simulink model "SingleStreamSSR"  (R2025a)
settings: Solver=VariableStepAuto  StartTime=0.0  StopTime=4096  RelTol=1e-3
PreLoadFcn:
  | xmcCheckSlxPath(bdroot)
  | SSR4_init
InitFcn:
  | xmcCheckSlxPath(bdroot)
  | SSR4_init;
values from neighbouring files (symbols this model uses):
  N = 512    [SSR4_init.m]
  SHIFT_ACC = 15    [SSR4_init.m]
  Taps = NormalizeCoef(UTaps,32768)    [SSR4_init.m]
undefined symbols (not defined in the file or in its folder): FIR_MultiKernel_cin, FIR_MultiKernel_cincout, FIR_MultiKernel_cout, S, SingleStream, vsva2197, xcvc1902
libraries: aieBasic x40, aieUtilities x8, dspobslib x1, simulink x1, vmcUtilities x1
(part 2 of 3)

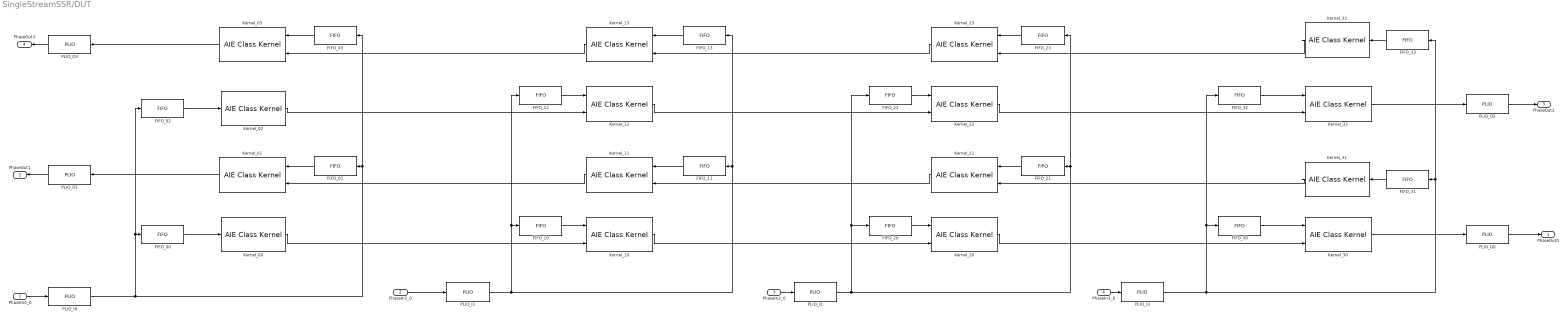
== system SingleStreamSSR/DUT ==
  PhaseIn0_0 : Inport
  PhaseIn1_0 : Inport  Port=2
  PhaseIn2_0 : Inport  Port=3
  PhaseIn3_0 : Inport  Port=4
  FIFO_00 : aieBasic/FIFO  FifoDepth=512  FIFOType=0  TileType=0  RowLocation=0  ColLocation=0  channel=0  blockJsonConstraints="[{\"type\":\"constraint\",\"constraintType\":\"location_fifo\",\"sid\":\"401\",\"lhs\":{\"type\":\"location\",\"templParam\":\"fifo\",\"args\":{\"type\":\"fifo\",\"name\":\"SingleStreamSSR/SSR4/FIFO_00\",\"sid\":\"401\"}},\"rhs\":{\"type\":\"fifogroup\",\"fifotype\":\"dma_fifo\",\"tiletype\":\"aie\",\"column\":{\"type\":\"evaluable\",\"expr\":\"25\",\"value\":25},\"row\":{\"type\":\"evaluable\",\"expr\":\"0\",\"value\":0},\"address\":{\"type\":\"evaluable\",\"expr\":\"0x0000\",\"value\":0},\"identifier\":\"0\",\"size\":{\"type\":\"evaluable\",\"expr\":\"512\",\"value\":512}},\"equality\":true}]"  deprecateConstraints=1
  FIFO_01 : aieBasic/FIFO  FifoDepth=512  FIFOType=0  TileType=0  RowLocation=0  ColLocation=0  channel=0  blockJsonConstraints="[{\"type\":\"constraint\",\"constraintType\":\"location_fifo\",\"sid\":\"404\",\"lhs\":{\"type\":\"location\",\"templParam\":\"fifo\",\"args\":{\"type\":\"fifo\",\"name\":\"SingleStreamSSR/SSR4/FIFO_01\",\"sid\":\"404\"}},\"rhs\":{\"type\":\"fifogroup\",\"fifotype\":\"dma_fifo\",\"tiletype\":\"aie\",\"column\":{\"type\":\"evaluable\",\"expr\":\"25\",\"value\":25},\"row\":{\"type\":\"evaluable\",\"expr\":\"1\",\"value\":1},\"address\":{\"type\":\"evaluable\",\"expr\":\"0x0000\",\"value\":0},\"identifier\":\"0\",\"size\":{\"type\":\"evaluable\",\"expr\":\"512\",\"value\":512}},\"equality\":true}]"  deprecateConstraints=1
  FIFO_02 : aieBasic/FIFO  FifoDepth=512  FIFOType=0  TileType=0  RowLocation=0  ColLocation=0  channel=0  blockJsonConstraints="[{\"type\":\"constraint\",\"constraintType\":\"location_fifo\",\"sid\":\"402\",\"lhs\":{\"type\":\"location\",\"templParam\":\"fifo\",\"args\":{\"type\":\"fifo\",\"name\":\"SingleStreamSSR/SSR4/FIFO_02\",\"sid\":\"402\"}},\"rhs\":{\"type\":\"fifogroup\",\"fifotype\":\"dma_fifo\",\"tiletype\":\"aie\",\"column\":{\"type\":\"evaluable\",\"expr\":\"25\",\"value\":25},\"row\":{\"type\":\"evaluable\",\"expr\":\"2\",\"value\":2},\"address\":{\"type\":\"evaluable\",\"expr\":\"0x0000\",\"value\":0},\"identifier\":\"0\",\"size\":{\"type\":\"evaluable\",\"expr\":\"512\",\"value\":512}},\"equality\":true}]"  deprecateConstraints=1
  FIFO_03 : aieBasic/FIFO  FifoDepth=512  FIFOType=0  TileType=0  RowLocation=0  ColLocation=0  channel=0  blockJsonConstraints="[{\"type\":\"constraint\",\"constraintType\":\"location_fifo\",\"sid\":\"403\",\"lhs\":{\"type\":\"location\",\"templParam\":\"fifo\",\"args\":{\"type\":\"fifo\",\"name\":\"SingleStreamSSR/SSR4/FIFO_03\",\"sid\":\"403\"}},\"rhs\":{\"type\":\"fifogroup\",\"fifotype\":\"dma_fifo\",\"tiletype\":\"aie\",\"column\":{\"type\":\"evaluable\",\"expr\":\"25\",\"value\":25},\"row\":{\"type\":\"evaluable\",\"expr\":\"3\",\"value\":3},\"address\":{\"type\":\"evaluable\",\"expr\":\"0x0000\",\"value\":0},\"identifier\":\"0\",\"size\":{\"type\":\"evaluable\",\"expr\":\"512\",\"value\":512}},\"equality\":true}]"  deprecateConstraints=1
  FIFO_10 : aieBasic/FIFO  FifoDepth=512  FIFOType=0  TileType=0  RowLocation=0  ColLocation=0  channel=0  blockJsonConstraints="[{\"type\":\"constraint\",\"constraintType\":\"location_fifo\",\"sid\":\"405\",\"lhs\":{\"type\":\"location\",\"templParam\":\"fifo\",\"args\":{\"type\":\"fifo\",\"name\":\"SingleStreamSSR/SSR4/FIFO_10\",\"sid\":\"405\"}},\"rhs\":{\"type\":\"fifogroup\",\"fifotype\":\"dma_fifo\",\"tiletype\":\"aie\",\"column\":{\"type\":\"evaluable\",\"expr\":\"26\",\"value\":26},\"row\":{\"type\":\"evaluable\",\"expr\":\"0\",\"value\":0},\"address\":{\"type\":\"evaluable\",\"expr\":\"0x0000\",\"value\":0},\"identifier\":\"0\",\"size\":{\"type\":\"evaluable\",\"expr\":\"512\",\"value\":512}},\"equality\":true}]"  deprecateConstraints=1
  FIFO_11 : aieBasic/FIFO  FifoDepth=512  FIFOType=0  TileType=0  RowLocation=0  ColLocation=0  channel=0  blockJsonConstraints="[{\"type\":\"constraint\",\"constraintType\":\"location_fifo\",\"sid\":\"407\",\"lhs\":{\"type\":\"location\",\"templParam\":\"fifo\",\"args\":{\"type\":\"fifo\",\"name\":\"SingleStreamSSR/SSR4/FIFO_11\",\"sid\":\"407\"}},\"rhs\":{\"type\":\"fifogroup\",\"fifotype\":\"dma_fifo\",\"tiletype\":\"aie\",\"column\":{\"type\":\"evaluable\",\"expr\":\"26\",\"value\":26},\"row\":{\"type\":\"evaluable\",\"expr\":\"1\",\"value\":1},\"address\":{\"type\":\"evaluable\",\"expr\":\"0x0000\",\"value\":0},\"identifier\":\"0\",\"size\":{\"type\":\"evaluable\",\"expr\":\"512\",\"value\":512}},\"equality\":true}]"  deprecateConstraints=1
  FIFO_12 : aieBasic/FIFO  FifoDepth=512  FIFOType=0  TileType=0  RowLocation=0  ColLocation=0  channel=0  blockJsonConstraints="[{\"type\":\"constraint\",\"constraintType\":\"location_fifo\",\"sid\":\"406\",\"lhs\":{\"type\":\"location\",\"templParam\":\"fifo\",\"args\":{\"type\":\"fifo\",\"name\":\"SingleStreamSSR/SSR4/FIFO_12\",\"sid\":\"406\"}},\"rhs\":{\"type\":\"fifogroup\",\"fifotype\":\"dma_fifo\",\"tiletype\":\"aie\",\"column\":{\"type\":\"evaluable\",\"expr\":\"26\",\"value\":26},\"row\":{\"type\":\"evaluable\",\"expr\":\"2\",\"value\":2},\"address\":{\"type\":\"evaluable\",\"expr\":\"0x0000\",\"value\":0},\"identifier\":\"0\",\"size\":{\"type\":\"evaluable\",\"expr\":\"512\",\"value\":512}},\"equality\":true}]"  deprecateConstraints=1
  FIFO_13 : aieBasic/FIFO  FifoDepth=512  FIFOType=0  TileType=0  RowLocation=0  ColLocation=0  channel=0  blockJsonConstraints="[{\"type\":\"constraint\",\"constraintType\":\"location_fifo\",\"sid\":\"408\",\"lhs\":{\"type\":\"location\",\"templParam\":\"fifo\",\"args\":{\"type\":\"fifo\",\"name\":\"SingleStreamSSR/SSR4/FIFO_13\",\"sid\":\"408\"}},\"rhs\":{\"type\":\"fifogroup\",\"fifotype\":\"dma_fifo\",\"tiletype\":\"aie\",\"column\":{\"type\":\"evaluable\",\"expr\":\"26\",\"value\":26},\"row\":{\"type\":\"evaluable\",\"expr\":\"3\",\"value\":3},\"address\":{\"type\":\"evaluable\",\"expr\":\"0x0000\",\"value\":0},\"identifier\":\"0\",\"size\":{\"type\":\"evaluable\",\"expr\":\"512\",\"value\":512}},\"equality\":true}]"  deprecateConstraints=1
  FIFO_20 : aieBasic/FIFO  FifoDepth=512  FIFOType=0  TileType=0  RowLocation=0  ColLocation=0  channel=0  blockJsonConstraints="[{\"type\":\"constraint\",\"constraintType\":\"location_fifo\",\"sid\":\"409\",\"lhs\":{\"type\":\"location\",\"templParam\":\"fifo\",\"args\":{\"type\":\"fifo\",\"name\":\"SingleStreamSSR/SSR4/FIFO_20\",\"sid\":\"409\"}},\"rhs\":{\"type\":\"fifogroup\",\"fifotype\":\"dma_fifo\",\"tiletype\":\"aie\",\"column\":{\"type\":\"evaluable\",\"expr\":\"27\",\"value\":27},\"row\":{\"type\":\"evaluable\",\"expr\":\"0\",\"value\":0},\"address\":{\"type\":\"evaluable\",\"expr\":\"0x0000\",\"value\":0},\"identifier\":\"0\",\"size\":{\"type\":\"evaluable\",\"expr\":\"512\",\"value\":512}},\"equality\":true}]"  deprecateConstraints=1
  FIFO_21 : aieBasic/FIFO  FifoDepth=512  FIFOType=0  TileType=0  RowLocation=0  ColLocation=0  channel=0  blockJsonConstraints="[{\"type\":\"constraint\",\"constraintType\":\"location_fifo\",\"sid\":\"412\",\"lhs\":{\"type\":\"location\",\"templParam\":\"fifo\",\"args\":{\"type\":\"fifo\",\"name\":\"SingleStreamSSR/SSR4/FIFO_21\",\"sid\":\"412\"}},\"rhs\":{\"type\":\"fifogroup\",\"fifotype\":\"dma_fifo\",\"tiletype\":\"aie\",\"column\":{\"type\":\"evaluable\",\"expr\":\"27\",\"value\":27},\"row\":{\"type\":\"evaluable\",\"expr\":\"1\",\"value\":1},\"address\":{\"type\":\"evaluable\",\"expr\":\"0x0000\",\"value\":0},\"identifier\":\"0\",\"size\":{\"type\":\"evaluable\",\"expr\":\"512\",\"value\":512}},\"equality\":true}]"  deprecateConstraints=1
  FIFO_22 : aieBasic/FIFO  FifoDepth=512  FIFOType=0  TileType=0  RowLocation=0  ColLocation=0  channel=0  blockJsonConstraints="[{\"type\":\"constraint\",\"constraintType\":\"location_fifo\",\"sid\":\"410\",\"lhs\":{\"type\":\"location\",\"templParam\":\"fifo\",\"args\":{\"type\":\"fifo\",\"name\":\"SingleStreamSSR/SSR4/FIFO_22\",\"sid\":\"410\"}},\"rhs\":{\"type\":\"fifogroup\",\"fifotype\":\"dma_fifo\",\"tiletype\":\"aie\",\"column\":{\"type\":\"evaluable\",\"expr\":\"27\",\"value\":27},\"row\":{\"type\":\"evaluable\",\"expr\":\"2\",\"value\":2},\"address\":{\"type\":\"evaluable\",\"expr\":\"0x0000\",\"value\":0},\"identifier\":\"0\",\"size\":{\"type\":\"evaluable\",\"expr\":\"512\",\"value\":512}},\"equality\":true}]"  deprecateConstraints=1
  FIFO_23 : aieBasic/FIFO  FifoDepth=512  FIFOType=0  TileType=0  RowLocation=0  ColLocation=0  channel=0  blockJsonConstraints="[{\"type\":\"constraint\",\"constraintType\":\"location_fifo\",\"sid\":\"411\",\"lhs\":{\"type\":\"location\",\"templParam\":\"fifo\",\"args\":{\"type\":\"fifo\",\"name\":\"SingleStreamSSR/SSR4/FIFO_23\",\"sid\":\"411\"}},\"rhs\":{\"type\":\"fifogroup\",\"fifotype\":\"dma_fifo\",\"tiletype\":\"aie\",\"column\":{\"type\":\"evaluable\",\"expr\":\"27\",\"value\":27},\"row\":{\"type\":\"evaluable\",\"expr\":\"3\",\"value\":3},\"address\":{\"type\":\"evaluable\",\"expr\":\"0x0000\",\"value\":0},\"identifier\":\"0\",\"size\":{\"type\":\"evaluable\",\"expr\":\"512\",\"value\":512}},\"equality\":true}]"  deprecateConstraints=1
  FIFO_30 : aieBasic/FIFO  FifoDepth=512  FIFOType=0  TileType=0  RowLocation=0  ColLocation=0  channel=0  blockJsonConstraints="[{\"type\":\"constraint\",\"constraintType\":\"location_fifo\",\"sid\":\"413\",\"lhs\":{\"type\":\"location\",\"templParam\":\"fifo\",\"args\":{\"type\":\"fifo\",\"name\":\"SingleStreamSSR/SSR4/FIFO_30\",\"sid\":\"413\"}},\"rhs\":{\"type\":\"fifogroup\",\"fifotype\":\"dma_fifo\",\"tiletype\":\"aie\",\"column\":{\"type\":\"evaluable\",\"expr\":\"28\",\"value\":28},\"row\":{\"type\":\"evaluable\",\"expr\":\"0\",\"value\":0},\"address\":{\"type\":\"evaluable\",\"expr\":\"0x0000\",\"value\":0},\"identifier\":\"0\",\"size\":{\"type\":\"evaluable\",\"expr\":\"512\",\"value\":512}},\"equality\":true}]"  deprecateConstraints=1
  FIFO_31 : aieBasic/FIFO  FifoDepth=512  FIFOType=0  TileType=0  RowLocation=0  ColLocation=0  channel=0  blockJsonConstraints="[{\"type\":\"constraint\",\"constraintType\":\"location_fifo\",\"sid\":\"416\",\"lhs\":{\"type\":\"location\",\"templParam\":\"fifo\",\"args\":{\"type\":\"fifo\",\"name\":\"SingleStreamSSR/SSR4/FIFO_31\",\"sid\":\"416\"}},\"rhs\":{\"type\":\"fifogroup\",\"fifotype\":\"dma_fifo\",\"tiletype\":\"aie\",\"column\":{\"type\":\"evaluable\",\"expr\":\"28\",\"value\":28},\"row\":{\"type\":\"evaluable\",\"expr\":\"1\",\"value\":1},\"address\":{\"type\":\"evaluable\",\"expr\":\"0x0000\",\"value\":0},\"identifier\":\"0\",\"size\":{\"type\":\"evaluable\",\"expr\":\"512\",\"value\":512}},\"equality\":true}]"  deprecateConstraints=1
  FIFO_32 : aieBasic/FIFO  FifoDepth=512  FIFOType=0  TileType=0  RowLocation=0  ColLocation=0  channel=0  blockJsonConstraints="[{\"type\":\"constraint\",\"constraintType\":\"location_fifo\",\"sid\":\"414\",\"lhs\":{\"type\":\"location\",\"templParam\":\"fifo\",\"args\":{\"type\":\"fifo\",\"name\":\"SingleStreamSSR/SSR4/FIFO_32\",\"sid\":\"414\"}},\"rhs\":{\"type\":\"fifogroup\",\"fifotype\":\"dma_fifo\",\"tiletype\":\"aie\",\"column\":{\"type\":\"evaluable\",\"expr\":\"28\",\"value\":28},\"row\":{\"type\":\"evaluable\",\"expr\":\"2\",\"value\":2},\"address\":{\"type\":\"evaluable\",\"expr\":\"0x0000\",\"value\":0},\"identifier\":\"0\",\"size\":{\"type\":\"evaluable\",\"expr\":\"512\",\"value\":512}},\"equality\":true}]"  deprecateConstraints=1
  FIFO_33 : aieBasic/FIFO  FifoDepth=512  FIFOType=0  TileType=0  RowLocation=0  ColLocation=0  channel=0  blockJsonConstraints="[{\"type\":\"constraint\",\"constraintType\":\"location_fifo\",\"sid\":\"415\",\"lhs\":{\"type\":\"location\",\"templParam\":\"fifo\",\"args\":{\"type\":\"fifo\",\"name\":\"SingleStreamSSR/SSR4/FIFO_33\",\"sid\":\"415\"}},\"rhs\":{\"type\":\"fifogroup\",\"fifotype\":\"dma_fifo\",\"tiletype\":\"aie\",\"column\":{\"type\":\"evaluable\",\"expr\":\"28\",\"value\":28},\"row\":{\"type\":\"evaluable\",\"expr\":\"3\",\"value\":3},\"address\":{\"type\":\"evaluable\",\"expr\":\"0x0000\",\"value\":0},\"identifier\":\"0\",\"size\":{\"type\":\"evaluable\",\"expr\":\"512\",\"value\":512}},\"equality\":true}]"  deprecateConstraints=1
  Kernel_00 : aieBasic/AIE Class Kernel  KernelAllAttrs=|  PortNames={'sin'; 'cout'}  PortSerializedTypes={'{P{Tinput_stream{1{t{Scint16}}}}}'; '{P{Toutput_cascade{2{t{Scacc48}}{t{Bv}}}}}'}  PortWindowSizes={0.000000000000000000e+00; 0.000000000000000000e+00}  PortWindowMargins={0.000000000000000000e+00; 0.000000000000000000e+00}  PortSynchronicities={'auto', 'auto'}  PortSignalSizes={0.000000000000000000e+00; 5.120000000000000000e+02}  ClassTemplateSpecKind=implicit  ClassTemplateParamNames={'NSamples'; 'ShiftAcc'}  ClassTemplateParamKinds={'nontype'; 'nontype'}  ClassTemplateParamTypes={'int'; 'int'}  ClassTemplateParamValues={'512', '15'}  ClassCtorParamNames={'taps'; 'Delay'}  ClassCtorParamSerializedTypes={'{R{Q1{C{Scint16}8}}}'; '{Q1{Bi32}}'}  ClassCtorParamValues={'[-54-21i -121-233i 102-525i 237-96i 8773-2748i 1454+497i 342+439i 14+121i]', '0'}  ClassIndex=1  ClassCtorIndex=1  ClassTabVisible=on  ClassTemplateParamsVisible=on  ClassCtorDeclVisible=on  ClassCtorParamsVisible=on  FunctionTabVisible=on  FunctionDecl=|  PortAttrs={ 'input', 'sin', 'input_stream_cint16 *', '', '0', '', ''; 'output', 'cout', 'output_cascade< cacc48, void > *', '', '', '', 'N' }  PortAttrsEnables={'off', 'off', 'off', 'off', 'off', 'off', 'off';'off', 'off', 'off', 'off', 'off', 'off', 'on'}  SampleTime=-1  ClassDeclTypeOptions=|  ClassDecl=|  ClassTemplateParams={ 'NSamples', 'int', 'BURST_LENGTH'; 'ShiftAcc', 'int', 'SHIFT_ACC' }  ClassTemplateParamsEnables={'off', 'off', 'on';'off', 'off', 'on'}  ClassCtorDeclTypeOptions=C[1 1]@t70@FIR_MultiKernel_cout(cint16 const ( & taps ) [ 8 ], int32 const Delay)  ClassCtorDecl=FIR_MultiKernel_cout(cint16 const ( & taps ) [ 8 ], int32 const Delay)  ClassCtorParams={ 'taps', 'cint16 const ( &) [ 8 ]', 'phi_0'; 'Delay', 'int32 const', '0' }  KernelHeaderFile=FirSingleStream.h  KernelClassName=SingleStream::FIR_MultiKernel_cout  KernelFunction=filter  KernelSourceFile=FirSingleStream.cpp  KernelSearchPaths={'$SRC', '$SRC/aie_kernels'}  PreProcOptions={}  blockJsonConstraints="{\"type\":\"constraint\",\"constraintType\":\"location_kernel\",\"sid\":\"386\",\"lhs\":{\"type\":\"location\",\"templParam\":\"kernel\",\"args\":{\"type\":\"kernel\",\"name\":\"SingleStreamSSR/SSR4/Kernel_00\",\"sid\":\"386\"}},\"rhs\":{\"type\":\"tile\",\"args\":[{\"type\":\"evaluable\",\"expr\":\"25\",\"value\":25},{\"type\":\"evaluable\",\"expr\":\"0\",\"value\":0}]},\"equality\":true}"
      KernelAllAttrs=|
      | s[12;12;9;9;19;14;21;23;21;23;24;21;15;17;12;24;26;26;26;27;28;9;21;23;23;23;24;25;14;19;19;29]@FunctionNameDeclFileNamePortNamesPortTypesPortSerializedTypesPortDirectionsPortWindowSizeEnablesPortWindowMarginEnablesPortBufferSizeEnablesPortBufferMarginEnablesPortSynchronicityEnablesPortSignalSizeEnablesPortBufferSizesPortBufferMarginsFunctionDeclFunctionTemplateSpecKindFunctionTemplateParamNamesFunctionTemplateParamKindsFunctionTemplateParamTypesFunctionTemplateParamValuesFunctionTemplateParamEnablesClassDeclClassTemplateSpecKindClassTemplateParamNamesClassTemplateParamKindsClassTemplateParamTypesClassTemplateParamValuesClassTemplateParamEnablesClassCtorDeclsClassCtorParamNamesClassCtorParamTypesClassCtorParamSerializedTypes[1 1]@C[32 1]@t6@filtert39@../../src/aie_kernels/FirSingleStream.hC[2 1]@t3@sint4@coutC[2 1]@t21@input_stream_cint16 *t32@output_cascade< cacc48, void > *C[2 1]@t33@{P{Tinput_stream{1{t{Scint16}}}}}t42@{P{Toutput_cascade{2{t{Scacc48}}{t{Bv}}}}}C[2 1]@t5@inputt6@outputC[2 1]@l0@l0@C[2 1]@l0@l0@C[2 1]@l0@l0@C[2 1]@l0@l0@C[2 1]@l0@l0@C[2 1]@l0@l1@C[2 1]@nnC[2 1]@nnt169@namespace SingleStream {
      | template < int NSamples, int ShiftAcc > 
      | void FIR_MultiKernel_cout::
      | filter(input_stream_cint16 * sin, output_cascade< cacc48, void > * cout);
      | }t4@nonee[0 1]@e[0 1]@e[0 1]@e[0 1]@e[0 1]@t94@namespace SingleStream {
      | template < int NSamples, int ShiftAcc > class FIR_MultiKernel_cout;
      | }t8@implicitC[2 1]@t8@NSamplest8@ShiftAccC[2 1]@t7@nontypet7@nontypeC[2 1]@t3@intt3@intC[2 1]@nnC[2 1]@l1@l1@C[1 1]@t70@FIR_MultiKernel_cout(cint16 const ( & taps ) [ 8 ], int32 const Delay)C[1 1]@C[2 1]@t4@tapst5@DelayC[1 1]@C[2 1]@t23@cint16 const ( &) [ 8 ]t11@int32 constC[1 1]@C[2 1]@t20@{R{Q1{C{Scint16}8}}}t10@{Q1{Bi32}}
      FunctionDecl=|
      | namespace SingleStream {
      | template < int NSamples, int ShiftAcc > 
      | void FIR_MultiKernel_cout::
      | filter(input_stream_cint16 * sin, output_cascade< cacc48, void > * cout);
      | }
      ClassDeclTypeOptions=|
      | C[1 1]@t94@namespace SingleStream {
      | template < int NSamples, int ShiftAcc > class FIR_MultiKernel_cout;
      | }
      ClassDecl=|
      | namespace SingleStream {
      | template < int NSamples, int ShiftAcc > class FIR_MultiKernel_cout;
      | }
  Kernel_01 : aieBasic/AIE Class Kernel  KernelAllAttrs=|  PortNames={'sin'; 'cin'; 'sout'}  PortSerializedTypes={'{P{Tinput_stream{1{t{Scint16}}}}}'; '{P{Tinput_cascade{2{t{Scacc48}}{t{Bv}}}}}'; '{P{Toutput_stream{1{t{Scint16}}}}}'}  PortWindowSizes={0.000000000000000000e+00; 0.000000000000000000e+00; 0.000000000000000000e+00}  PortWindowMargins={0.000000000000000000e+00; 0.000000000000000000e+00; 0.000000000000000000e+00}  PortSynchronicities={'auto', 'auto', 'auto'}  PortSignalSizes={0.000000000000000000e+00; 0.000000000000000000e+00; 5.120000000000000000e+02}  ClassTemplateSpecKind=implicit  ClassTemplateParamNames={'NSamples'; 'ShiftAcc'}  ClassTemplateParamKinds={'nontype'; 'nontype'}  ClassTemplateParamTypes={'int'; 'int'}  ClassTemplateParamValues={'512', '15'}  ClassCtorParamNames={'taps'; 'Delay'}  ClassCtorParamSerializedTypes={'{R{Q1{C{Scint16}8}}}'; '{Q1{Bi32}}'}  ClassCtorParamValues={'[14-121i 342-439i 1454-497i 8773+2748i 237+96i 102+525i -121+233i -54+21i]', '1'}  ClassIndex=1  ClassCtorIndex=1  ClassTabVisible=on  ClassTemplateParamsVisible=on  ClassCtorDeclVisible=on  ClassCtorParamsVisible=on  FunctionTabVisible=on  FunctionDecl=|  PortAttrs={ 'input', 'sin', 'input_stream_cint16 *', '', '0', '', ''; 'input', 'cin', 'input_cascade< cacc48, void > *', '', '0', '', ''; 'output', 'sout', 'output_stream_cint16 *', '', '', '', 'N' }  PortAttrsEnables={'off', 'off', 'off', 'off', 'off', 'off', 'off';'off', 'off', 'off', 'off', 'off', 'off', 'off';'off', 'off', 'off', 'off', 'off', 'off', 'on'}  SampleTime=-1  ClassDeclTypeOptions=|  ClassDecl=|  ClassTemplateParams={ 'NSamples', 'int', 'BURST_LENGTH'; 'ShiftAcc', 'int', 'SHIFT_ACC' }  ClassTemplateParamsEnables={'off', 'off', 'on';'off', 'off', 'on'}  ClassCtorDeclTypeOptions=C[1 1]@t69@FIR_MultiKernel_cin(cint16 const ( & taps ) [ 8 ], int32 const Delay)  ClassCtorDecl=FIR_MultiKernel_cin(cint16 const ( & taps ) [ 8 ], int32 const Delay)  ClassCtorParams={ 'taps', 'cint16 const ( &) [ 8 ]', 'phi_3'; 'Delay', 'int32 const', '1' }  KernelHeaderFile=FirSingleStream.h  KernelClassName=SingleStream::FIR_MultiKernel_cin  KernelFunction=filter  KernelSourceFile=FirSingleStream.cpp  KernelSearchPaths={'$SRC', '$SRC/aie_kernels'}  PreProcOptions={}  blockJsonConstraints=[]
      KernelAllAttrs=|
      | s[12;12;9;9;19;14;21;23;21;23;24;21;15;17;12;24;26;26;26;27;28;9;21;23;23;23;24;25;14;19;19;29]@FunctionNameDeclFileNamePortNamesPortTypesPortSerializedTypesPortDirectionsPortWindowSizeEnablesPortWindowMarginEnablesPortBufferSizeEnablesPortBufferMarginEnablesPortSynchronicityEnablesPortSignalSizeEnablesPortBufferSizesPortBufferMarginsFunctionDeclFunctionTemplateSpecKindFunctionTemplateParamNamesFunctionTemplateParamKindsFunctionTemplateParamTypesFunctionTemplateParamValuesFunctionTemplateParamEnablesClassDeclClassTemplateSpecKindClassTemplateParamNamesClassTemplateParamKindsClassTemplateParamTypesClassTemplateParamValuesClassTemplateParamEnablesClassCtorDeclsClassCtorParamNamesClassCtorParamTypesClassCtorParamSerializedTypes[1 1]@C[32 1]@t6@filtert39@../../src/aie_kernels/FirSingleStream.hC[3 1]@t3@sint3@cint4@soutC[3 1]@t21@input_stream_cint16 *t31@input_cascade< cacc48, void > *t22@output_stream_cint16 *C[3 1]@t33@{P{Tinput_stream{1{t{Scint16}}}}}t41@{P{Tinput_cascade{2{t{Scacc48}}{t{Bv}}}}}t34@{P{Toutput_stream{1{t{Scint16}}}}}C[3 1]@t5@inputt5@inputt6@outputC[3 1]@l0@l0@l0@C[3 1]@l0@l0@l0@C[3 1]@l0@l0@l0@C[3 1]@l0@l0@l0@C[3 1]@l0@l0@l0@C[3 1]@l0@l0@l1@C[3 1]@nnnC[3 1]@nnnt195@namespace SingleStream {
      | template < int NSamples, int ShiftAcc > 
      | void FIR_MultiKernel_cin::
      | filter(input_stream_cint16 * sin, input_cascade< cacc48, void > * cin, output_stream_cint16 * sout);
      | }t4@nonee[0 1]@e[0 1]@e[0 1]@e[0 1]@e[0 1]@t93@namespace SingleStream {
      | template < int NSamples, int ShiftAcc > class FIR_MultiKernel_cin;
      | }t8@implicitC[2 1]@t8@NSamplest8@ShiftAccC[2 1]@t7@nontypet7@nontypeC[2 1]@t3@intt3@intC[2 1]@nnC[2 1]@l1@l1@C[1 1]@t69@FIR_MultiKernel_cin(cint16 const ( & taps ) [ 8 ], int32 const Delay)C[1 1]@C[2 1]@t4@tapst5@DelayC[1 1]@C[2 1]@t23@cint16 const ( &) [ 8 ]t11@int32 constC[1 1]@C[2 1]@t20@{R{Q1{C{Scint16}8}}}t10@{Q1{Bi32}}
      FunctionDecl=|
      | namespace SingleStream {
      | template < int NSamples, int ShiftAcc > 
      | void FIR_MultiKernel_cin::
      | filter(input_stream_cint16 * sin, input_cascade< cacc48, void > * cin, output_stream_cint16 * sout);
      | }
      ClassDeclTypeOptions=|
      | C[1 1]@t93@namespace SingleStream {
      | template < int NSamples, int ShiftAcc > class FIR_MultiKernel_cin;
      | }
      ClassDecl=|
      | namespace SingleStream {
      | template < int NSamples, int ShiftAcc > class FIR_MultiKernel_cin;
      | }
  Kernel_02 : aieBasic/AIE Class Kernel  KernelAllAttrs=|  PortNames={'sin'; 'cout'}  PortSerializedTypes={'{P{Tinput_stream{1{t{Scint16}}}}}'; '{P{Toutput_cascade{2{t{Scacc48}}{t{Bv}}}}}'}  PortWindowSizes={0.000000000000000000e+00; 0.000000000000000000e+00}  PortWindowMargins={0.000000000000000000e+00; 0.000000000000000000e+00}  PortSynchronicities={'auto', 'auto'}  PortSignalSizes={0.000000000000000000e+00; 5.120000000000000000e+02}  ClassTemplateSpecKind=implicit  ClassTemplateParamNames={'NSamples'; 'ShiftAcc'}  ClassTemplateParamKinds={'nontype'; 'nontype'}  ClassTemplateParamTypes={'int'; 'int'}  ClassTemplateParamValues={'512', '15'}  ClassCtorParamNames={'taps'; 'Delay'}  ClassCtorParamSerializedTypes={'{R{Q1{C{Scint16}8}}}'; '{Q1{Bi32}}'}  ClassCtorParamValues={'[-21+26i 146-91i 1183+239i 4086+5221i 248-2878i 237-54i -160+111i -83-21i]', '1'}  ClassIndex=1  ClassCtorIndex=1  ClassTabVisible=on  ClassTemplateParamsVisible=on  ClassCtorDeclVisible=on  ClassCtorParamsVisible=on  FunctionTabVisible=on  FunctionDecl=|  PortAttrs={ 'input', 'sin', 'input_stream_cint16 *', '', '0', '', ''; 'output', 'cout', 'output_cascade< cacc48, void > *', '', '', '', 'N' }  PortAttrsEnables={'off', 'off', 'off', 'off', 'off', 'off', 'off';'off', 'off', 'off', 'off', 'off', 'off', 'on'}  SampleTime=-1  ClassDeclTypeOptions=|  ClassDecl=|  ClassTemplateParams={ 'NSamples', 'int', 'BURST_LENGTH'; 'ShiftAcc', 'int', 'SHIFT_ACC' }  ClassTemplateParamsEnables={'off', 'off', 'on';'off', 'off', 'on'}  ClassCtorDeclTypeOptions=C[1 1]@t70@FIR_MultiKernel_cout(cint16 const ( & taps ) [ 8 ], int32 const Delay)  ClassCtorDecl=FIR_MultiKernel_cout(cint16 const ( & taps ) [ 8 ], int32 const Delay)  ClassCtorParams={ 'taps', 'cint16 const ( &) [ 8 ]', 'phi_2'; 'Delay', 'int32 const', '1' }  KernelHeaderFile=FirSingleStream.h  KernelClassName=SingleStream::FIR_MultiKernel_cout  KernelFunction=filter  KernelSourceFile=FirSingleStream.cpp  KernelSearchPaths={'$SRC', '$SRC/aie_kernels'}  PreProcOptions={}  blockJsonConstraints="{\"type\":\"constraint\",\"constraintType\":\"location_kernel\",\"sid\":\"341\",\"lhs\":{\"type\":\"location\",\"templParam\":\"kernel\",\"args\":{\"type\":\"kernel\",\"name\":\"SingleStreamSSR/SSR4/Kernel_02\",\"sid\":\"341\"}},\"rhs\":{\"type\":\"tile\",\"args\":[{\"type\":\"evaluable\",\"expr\":\"25\",\"value\":25},{\"type\":\"evaluable\",\"expr\":\"2\",\"value\":2}]},\"equality\":true}"
      KernelAllAttrs=|
      | s[12;12;9;9;19;14;21;23;21;23;24;21;15;17;12;24;26;26;26;27;28;9;21;23;23;23;24;25;14;19;19;29]@FunctionNameDeclFileNamePortNamesPortTypesPortSerializedTypesPortDirectionsPortWindowSizeEnablesPortWindowMarginEnablesPortBufferSizeEnablesPortBufferMarginEnablesPortSynchronicityEnablesPortSignalSizeEnablesPortBufferSizesPortBufferMarginsFunctionDeclFunctionTemplateSpecKindFunctionTemplateParamNamesFunctionTemplateParamKindsFunctionTemplateParamTypesFunctionTemplateParamValuesFunctionTemplateParamEnablesClassDeclClassTemplateSpecKindClassTemplateParamNamesClassTemplateParamKindsClassTemplateParamTypesClassTemplateParamValuesClassTemplateParamEnablesClassCtorDeclsClassCtorParamNamesClassCtorParamTypesClassCtorParamSerializedTypes[1 1]@C[32 1]@t6@filtert39@../../src/aie_kernels/FirSingleStream.hC[2 1]@t3@sint4@coutC[2 1]@t21@input_stream_cint16 *t32@output_cascade< cacc48, void > *C[2 1]@t33@{P{Tinput_stream{1{t{Scint16}}}}}t42@{P{Toutput_cascade{2{t{Scacc48}}{t{Bv}}}}}C[2 1]@t5@inputt6@outputC[2 1]@l0@l0@C[2 1]@l0@l0@C[2 1]@l0@l0@C[2 1]@l0@l0@C[2 1]@l0@l0@C[2 1]@l0@l1@C[2 1]@nnC[2 1]@nnt169@namespace SingleStream {
      | template < int NSamples, int ShiftAcc > 
      | void FIR_MultiKernel_cout::
      | filter(input_stream_cint16 * sin, output_cascade< cacc48, void > * cout);
      | }t4@nonee[0 1]@e[0 1]@e[0 1]@e[0 1]@e[0 1]@t94@namespace SingleStream {
      | template < int NSamples, int ShiftAcc > class FIR_MultiKernel_cout;
      | }t8@implicitC[2 1]@t8@NSamplest8@ShiftAccC[2 1]@t7@nontypet7@nontypeC[2 1]@t3@intt3@intC[2 1]@nnC[2 1]@l1@l1@C[1 1]@t70@FIR_MultiKernel_cout(cint16 const ( & taps ) [ 8 ], int32 const Delay)C[1 1]@C[2 1]@t4@tapst5@DelayC[1 1]@C[2 1]@t23@cint16 const ( &) [ 8 ]t11@int32 constC[1 1]@C[2 1]@t20@{R{Q1{C{Scint16}8}}}t10@{Q1{Bi32}}
      FunctionDecl=|
      | namespace SingleStream {
      | template < int NSamples, int ShiftAcc > 
      | void FIR_MultiKernel_cout::
      | filter(input_stream_cint16 * sin, output_cascade< cacc48, void > * cout);
      | }
      ClassDeclTypeOptions=|
      | C[1 1]@t94@namespace SingleStream {
      | template < int NSamples, int ShiftAcc > class FIR_MultiKernel_cout;
      | }
      ClassDecl=|
      | namespace SingleStream {
      | template < int NSamples, int ShiftAcc > class FIR_MultiKernel_cout;
      | }
  Kernel_03 : aieBasic/AIE Class Kernel  KernelAllAttrs=|  PortNames={'sin'; 'cin'; 'sout'}  PortSerializedTypes={'{P{Tinput_stream{1{t{Scint16}}}}}'; '{P{Tinput_cascade{2{t{Scacc48}}{t{Bv}}}}}'; '{P{Toutput_stream{1{t{Scint16}}}}}'}  PortWindowSizes={0.000000000000000000e+00; 0.000000000000000000e+00; 0.000000000000000000e+00}  PortWindowMargins={0.000000000000000000e+00; 0.000000000000000000e+00; 0.000000000000000000e+00}  PortSynchronicities={'auto', 'auto', 'auto'}  PortSignalSizes={0.000000000000000000e+00; 0.000000000000000000e+00; 5.120000000000000000e+02}  ClassTemplateSpecKind=implicit  ClassTemplateParamNames={'NSamples'; 'ShiftAcc'}  ClassTemplateParamKinds={'nontype'; 'nontype'}  ClassTemplateParamTypes={'int'; 'int'}  ClassTemplateParamValues={'512', '15'}  ClassCtorParamNames={'taps'; 'Delay'}  ClassCtorParamSerializedTypes={'{R{Q1{C{Scint16}8}}}'; '{Q1{Bi32}}'}  ClassCtorParamValues={'[-83+21i -160-111i 237+54i 248+2878i 4086-5221i 1183-239i 146+91i -21-26i]', '1'}  ClassIndex=1  ClassCtorIndex=1  ClassTabVisible=on  ClassTemplateParamsVisible=on  ClassCtorDeclVisible=on  ClassCtorParamsVisible=on  FunctionTabVisible=on  FunctionDecl=|  PortAttrs={ 'input', 'sin', 'input_stream_cint16 *', '', '0', '', ''; 'input', 'cin', 'input_cascade< cacc48, void > *', '', '0', '', ''; 'output', 'sout', 'output_stream_cint16 *', '', '', '', 'N' }  PortAttrsEnables={'off', 'off', 'off', 'off', 'off', 'off', 'off';'off', 'off', 'off', 'off', 'off', 'off', 'off';'off', 'off', 'off', 'off', 'off', 'off', 'on'}  SampleTime=-1  ClassDeclTypeOptions=|  ClassDecl=|  ClassTemplateParams={ 'NSamples', 'int', 'BURST_LENGTH'; 'ShiftAcc', 'int', 'SHIFT_ACC' }  ClassTemplateParamsEnables={'off', 'off', 'on';'off', 'off', 'on'}  ClassCtorDeclTypeOptions=C[1 1]@t69@FIR_MultiKernel_cin(cint16 const ( & taps ) [ 8 ], int32 const Delay)  ClassCtorDecl=FIR_MultiKernel_cin(cint16 const ( & taps ) [ 8 ], int32 const Delay)  ClassCtorParams={ 'taps', 'cint16 const ( &) [ 8 ]', 'phi_1'; 'Delay', 'int32 const', '1' }  KernelHeaderFile=FirSingleStream.h  KernelClassName=SingleStream::FIR_MultiKernel_cin  KernelFunction=filter  KernelSourceFile=FirSingleStream.cpp  KernelSearchPaths={'$SRC', '$SRC/aie_kernels'}  PreProcOptions={}  blockJsonConstraints=[]
      KernelAllAttrs=|
      | s[12;12;9;9;19;14;21;23;21;23;24;21;15;17;12;24;26;26;26;27;28;9;21;23;23;23;24;25;14;19;19;29]@FunctionNameDeclFileNamePortNamesPortTypesPortSerializedTypesPortDirectionsPortWindowSizeEnablesPortWindowMarginEnablesPortBufferSizeEnablesPortBufferMarginEnablesPortSynchronicityEnablesPortSignalSizeEnablesPortBufferSizesPortBufferMarginsFunctionDeclFunctionTemplateSpecKindFunctionTemplateParamNamesFunctionTemplateParamKindsFunctionTemplateParamTypesFunctionTemplateParamValuesFunctionTemplateParamEnablesClassDeclClassTemplateSpecKindClassTemplateParamNamesClassTemplateParamKindsClassTemplateParamTypesClassTemplateParamValuesClassTemplateParamEnablesClassCtorDeclsClassCtorParamNamesClassCtorParamTypesClassCtorParamSerializedTypes[1 1]@C[32 1]@t6@filtert39@../../src/aie_kernels/FirSingleStream.hC[3 1]@t3@sint3@cint4@soutC[3 1]@t21@input_stream_cint16 *t31@input_cascade< cacc48, void > *t22@output_stream_cint16 *C[3 1]@t33@{P{Tinput_stream{1{t{Scint16}}}}}t41@{P{Tinput_cascade{2{t{Scacc48}}{t{Bv}}}}}t34@{P{Toutput_stream{1{t{Scint16}}}}}C[3 1]@t5@inputt5@inputt6@outputC[3 1]@l0@l0@l0@C[3 1]@l0@l0@l0@C[3 1]@l0@l0@l0@C[3 1]@l0@l0@l0@C[3 1]@l0@l0@l0@C[3 1]@l0@l0@l1@C[3 1]@nnnC[3 1]@nnnt195@namespace SingleStream {
      | template < int NSamples, int ShiftAcc > 
      | void FIR_MultiKernel_cin::
      | filter(input_stream_cint16 * sin, input_cascade< cacc48, void > * cin, output_stream_cint16 * sout);
      | }t4@nonee[0 1]@e[0 1]@e[0 1]@e[0 1]@e[0 1]@t93@namespace SingleStream {
      | template < int NSamples, int ShiftAcc > class FIR_MultiKernel_cin;
      | }t8@implicitC[2 1]@t8@NSamplest8@ShiftAccC[2 1]@t7@nontypet7@nontypeC[2 1]@t3@intt3@intC[2 1]@nnC[2 1]@l1@l1@C[1 1]@t69@FIR_MultiKernel_cin(cint16 const ( & taps ) [ 8 ], int32 const Delay)C[1 1]@C[2 1]@t4@tapst5@DelayC[1 1]@C[2 1]@t23@cint16 const ( &) [ 8 ]t11@int32 constC[1 1]@C[2 1]@t20@{R{Q1{C{Scint16}8}}}t10@{Q1{Bi32}}
      FunctionDecl=|
      | namespace SingleStream {
      | template < int NSamples, int ShiftAcc > 
      | void FIR_MultiKernel_cin::
      | filter(input_stream_cint16 * sin, input_cascade< cacc48, void > * cin, output_stream_cint16 * sout);
      | }
      ClassDeclTypeOptions=|
      | C[1 1]@t93@namespace SingleStream {
      | template < int NSamples, int ShiftAcc > class FIR_MultiKernel_cin;
      | }
      ClassDecl=|
      | namespace SingleStream {
      | template < int NSamples, int ShiftAcc > class FIR_MultiKernel_cin;
      | }
  Kernel_10 : aieBasic/AIE Class Kernel  KernelAllAttrs=|  PortNames={'sin'; 'cin'; 'cout'}  PortSerializedTypes={'{P{Tinput_stream{1{t{Scint16}}}}}'; '{P{Tinput_cascade{2{t{Scacc48}}{t{Bv}}}}}'; '{P{Toutput_cascade{2{t{Scacc48}}{t{Bv}}}}}'}  PortWindowSizes={0.000000000000000000e+00; 0.000000000000000000e+00; 0.000000000000000000e+00}  PortWindowMargins={0.000000000000000000e+00; 0.000000000000000000e+00; 0.000000000000000000e+00}  PortSynchronicities={'auto', 'auto', 'auto'}  PortSignalSizes={0.000000000000000000e+00; 0.000000000000000000e+00; 5.120000000000000000e+02}  ClassTemplateSpecKind=implicit  ClassTemplateParamNames={'NSamples'; 'ShiftAcc'}  ClassTemplateParamKinds={'nontype'; 'nontype'}  ClassTemplateParamTypes={'int'; 'int'}  ClassTemplateParamValues={'512', '15'}  ClassCtorParamNames={'taps'; 'Delay'}  ClassCtorParamSerializedTypes={'{R{Q1{C{Scint16}8}}}'; '{Q1{Bi32}}'}  ClassCtorParamValues={'[-83+21i -160-111i 237+54i 248+2878i 4086-5221i 1183-239i 146+91i -21-26i]', '0'}  ClassIndex=1  ClassCtorIndex=1  ClassTabVisible=on  ClassTemplateParamsVisible=on  ClassCtorDeclVisible=on  ClassCtorParamsVisible=on  FunctionTabVisible=on  FunctionDecl=|  PortAttrs={ 'input', 'sin', 'input_stream_cint16 *', '', '0', '', ''; 'input', 'cin', 'input_cascade< cacc48, void > *', '', '0', '', ''; 'output', 'cout', 'output_cascade< cacc48, void > *', '', '', '', 'N' }  PortAttrsEnables={'off', 'off', 'off', 'off', 'off', 'off', 'off';'off', 'off', 'off', 'off', 'off', 'off', 'off';'off', 'off', 'off', 'off', 'off', 'off', 'on'}  SampleTime=-1  ClassDeclTypeOptions=|  ClassDecl=|  ClassTemplateParams={ 'NSamples', 'int', 'BURST_LENGTH'; 'ShiftAcc', 'int', 'SHIFT_ACC' }  ClassTemplateParamsEnables={'off', 'off', 'on';'off', 'off', 'on'}  ClassCtorDeclTypeOptions=C[1 1]@t73@FIR_MultiKernel_cincout(cint16 const ( & taps ) [ 8 ], int32 const Delay)  ClassCtorDecl=FIR_MultiKernel_cincout(cint16 const ( & taps ) [ 8 ], int32 const Delay)  ClassCtorParams={ 'taps', 'cint16 const ( &) [ 8 ]', 'phi_1'; 'Delay', 'int32 const', '0' }  KernelHeaderFile=FirSingleStream.h  KernelClassName=SingleStream::FIR_MultiKernel_cincout  KernelFunction=filter  KernelSourceFile=FirSingleStream.cpp  KernelSearchPaths={'$SRC', '$SRC/aie_kernels'}  PreProcOptions={}  blockJsonConstraints=[]
      KernelAllAttrs=|
      | s[12;12;9;9;19;14;21;23;21;23;24;21;15;17;12;24;26;26;26;27;28;9;21;23;23;23;24;25;14;19;19;29]@FunctionNameDeclFileNamePortNamesPortTypesPortSerializedTypesPortDirectionsPortWindowSizeEnablesPortWindowMarginEnablesPortBufferSizeEnablesPortBufferMarginEnablesPortSynchronicityEnablesPortSignalSizeEnablesPortBufferSizesPortBufferMarginsFunctionDeclFunctionTemplateSpecKindFunctionTemplateParamNamesFunctionTemplateParamKindsFunctionTemplateParamTypesFunctionTemplateParamValuesFunctionTemplateParamEnablesClassDeclClassTemplateSpecKindClassTemplateParamNamesClassTemplateParamKindsClassTemplateParamTypesClassTemplateParamValuesClassTemplateParamEnablesClassCtorDeclsClassCtorParamNamesClassCtorParamTypesClassCtorParamSerializedTypes[1 1]@C[32 1]@t6@filtert39@../../src/aie_kernels/FirSingleStream.hC[3 1]@t3@sint3@cint4@coutC[3 1]@t21@input_stream_cint16 *t31@input_cascade< cacc48, void > *t32@output_cascade< cacc48, void > *C[3 1]@t33@{P{Tinput_stream{1{t{Scint16}}}}}t41@{P{Tinput_cascade{2{t{Scacc48}}{t{Bv}}}}}t42@{P{Toutput_cascade{2{t{Scacc48}}{t{Bv}}}}}C[3 1]@t5@inputt5@inputt6@outputC[3 1]@l0@l0@l0@C[3 1]@l0@l0@l0@C[3 1]@l0@l0@l0@C[3 1]@l0@l0@l0@C[3 1]@l0@l0@l0@C[3 1]@l0@l0@l1@C[3 1]@nnnC[3 1]@nnnt209@namespace SingleStream {
      | template < int NSamples, int ShiftAcc > 
      | void FIR_MultiKernel_cincout::
      | filter(input_stream_cint16 * sin, input_cascade< cacc48, void > * cin, output_cascade< cacc48, void > * cout);
      | }t4@nonee[0 1]@e[0 1]@e[0 1]@e[0 1]@e[0 1]@t97@namespace SingleStream {
      | template < int NSamples, int ShiftAcc > class FIR_MultiKernel_cincout;
      | }t8@implicitC[2 1]@t8@NSamplest8@ShiftAccC[2 1]@t7@nontypet7@nontypeC[2 1]@t3@intt3@intC[2 1]@nnC[2 1]@l1@l1@C[1 1]@t73@FIR_MultiKernel_cincout(cint16 const ( & taps ) [ 8 ], int32 const Delay)C[1 1]@C[2 1]@t4@tapst5@DelayC[1 1]@C[2 1]@t23@cint16 const ( &) [ 8 ]t11@int32 constC[1 1]@C[2 1]@t20@{R{Q1{C{Scint16}8}}}t10@{Q1{Bi32}}
      FunctionDecl=|
      | namespace SingleStream {
      | template < int NSamples, int ShiftAcc > 
      | void FIR_MultiKernel_cincout::
      | filter(input_stream_cint16 * sin, input_cascade< cacc48, void > * cin, output_cascade< cacc48, void > * cout);
      | }
      ClassDeclTypeOptions=|
      | C[1 1]@t97@namespace SingleStream {
      | template < int NSamples, int ShiftAcc > class FIR_MultiKernel_cincout;
      | }
      ClassDecl=|
      | namespace SingleStream {
      | template < int NSamples, int ShiftAcc > class FIR_MultiKernel_cincout;
      | }
  Kernel_11 : aieBasic/AIE Class Kernel  KernelAllAttrs=|  PortNames={'sin'; 'cin'; 'cout'}  PortSerializedTypes={'{P{Tinput_stream{1{t{Scint16}}}}}'; '{P{Tinput_cascade{2{t{Scacc48}}{t{Bv}}}}}'; '{P{Toutput_cascade{2{t{Scacc48}}{t{Bv}}}}}'}  PortWindowSizes={0.000000000000000000e+00; 0.000000000000000000e+00; 0.000000000000000000e+00}  PortWindowMargins={0.000000000000000000e+00; 0.000000000000000000e+00; 0.000000000000000000e+00}  PortSynchronicities={'auto', 'auto', 'auto'}  PortSignalSizes={0.000000000000000000e+00; 0.000000000000000000e+00; 5.120000000000000000e+02}  ClassTemplateSpecKind=implicit  ClassTemplateParamNames={'NSamples'; 'ShiftAcc'}  ClassTemplateParamKinds={'nontype'; 'nontype'}  ClassTemplateParamTypes={'int'; 'int'}  ClassTemplateParamValues={'512', '15'}  ClassCtorParamNames={'taps'; 'Delay'}  ClassCtorParamSerializedTypes={'{R{Q1{C{Scint16}8}}}'; '{Q1{Bi32}}'}  ClassCtorParamValues={'[-54-21i -121-233i 102-525i 237-96i 8773-2748i 1454+497i 342+439i 14+121i]', '0'}  ClassIndex=1  ClassCtorIndex=1  ClassTabVisible=on  ClassTemplateParamsVisible=on  ClassCtorDeclVisible=on  ClassCtorParamsVisible=on  FunctionTabVisible=on  FunctionDecl=|  PortAttrs={ 'input', 'sin', 'input_stream_cint16 *', '', '0', '', ''; 'input', 'cin', 'input_cascade< cacc48, void > *', '', '0', '', ''; 'output', 'cout', 'output_cascade< cacc48, void > *', '', '', '', 'N' }  PortAttrsEnables={'off', 'off', 'off', 'off', 'off', 'off', 'off';'off', 'off', 'off', 'off', 'off', 'off', 'off';'off', 'off', 'off', 'off', 'off', 'off', 'on'}  SampleTime=-1  ClassDeclTypeOptions=|  ClassDecl=|  ClassTemplateParams={ 'NSamples', 'int', 'BURST_LENGTH'; 'ShiftAcc', 'int', 'SHIFT_ACC' }  ClassTemplateParamsEnables={'off', 'off', 'on';'off', 'off', 'on'}  ClassCtorDeclTypeOptions=C[1 1]@t73@FIR_MultiKernel_cincout(cint16 const ( & taps ) [ 8 ], int32 const Delay)  ClassCtorDecl=FIR_MultiKernel_cincout(cint16 const ( & taps ) [ 8 ], int32 const Delay)  ClassCtorParams={ 'taps', 'cint16 const ( &) [ 8 ]', 'phi_0'; 'Delay', 'int32 const', '0' }  KernelHeaderFile=FirSingleStream.h  KernelClassName=SingleStream::FIR_MultiKernel_cincout  KernelFunction=filter  KernelSourceFile=FirSingleStream.cpp  KernelSearchPaths={'$SRC', '$SRC/aie_kernels'}  PreProcOptions={}  blockJsonConstraints=[]
      KernelAllAttrs=|
      | s[12;12;9;9;19;14;21;23;21;23;24;21;15;17;12;24;26;26;26;27;28;9;21;23;23;23;24;25;14;19;19;29]@FunctionNameDeclFileNamePortNamesPortTypesPortSerializedTypesPortDirectionsPortWindowSizeEnablesPortWindowMarginEnablesPortBufferSizeEnablesPortBufferMarginEnablesPortSynchronicityEnablesPortSignalSizeEnablesPortBufferSizesPortBufferMarginsFunctionDeclFunctionTemplateSpecKindFunctionTemplateParamNamesFunctionTemplateParamKindsFunctionTemplateParamTypesFunctionTemplateParamValuesFunctionTemplateParamEnablesClassDeclClassTemplateSpecKindClassTemplateParamNamesClassTemplateParamKindsClassTemplateParamTypesClassTemplateParamValuesClassTemplateParamEnablesClassCtorDeclsClassCtorParamNamesClassCtorParamTypesClassCtorParamSerializedTypes[1 1]@C[32 1]@t6@filtert39@../../src/aie_kernels/FirSingleStream.hC[3 1]@t3@sint3@cint4@coutC[3 1]@t21@input_stream_cint16 *t31@input_cascade< cacc48, void > *t32@output_cascade< cacc48, void > *C[3 1]@t33@{P{Tinput_stream{1{t{Scint16}}}}}t41@{P{Tinput_cascade{2{t{Scacc48}}{t{Bv}}}}}t42@{P{Toutput_cascade{2{t{Scacc48}}{t{Bv}}}}}C[3 1]@t5@inputt5@inputt6@outputC[3 1]@l0@l0@l0@C[3 1]@l0@l0@l0@C[3 1]@l0@l0@l0@C[3 1]@l0@l0@l0@C[3 1]@l0@l0@l0@C[3 1]@l0@l0@l1@C[3 1]@nnnC[3 1]@nnnt209@namespace SingleStream {
      | template < int NSamples, int ShiftAcc > 
      | void FIR_MultiKernel_cincout::
      | filter(input_stream_cint16 * sin, input_cascade< cacc48, void > * cin, output_cascade< cacc48, void > * cout);
      | }t4@nonee[0 1]@e[0 1]@e[0 1]@e[0 1]@e[0 1]@t97@namespace SingleStream {
      | template < int NSamples, int ShiftAcc > class FIR_MultiKernel_cincout;
      | }t8@implicitC[2 1]@t8@NSamplest8@ShiftAccC[2 1]@t7@nontypet7@nontypeC[2 1]@t3@intt3@intC[2 1]@nnC[2 1]@l1@l1@C[1 1]@t73@FIR_MultiKernel_cincout(cint16 const ( & taps ) [ 8 ], int32 const Delay)C[1 1]@C[2 1]@t4@tapst5@DelayC[1 1]@C[2 1]@t23@cint16 const ( &) [ 8 ]t11@int32 constC[1 1]@C[2 1]@t20@{R{Q1{C{Scint16}8}}}t10@{Q1{Bi32}}
      FunctionDecl=|
      | namespace SingleStream {
      | template < int NSamples, int ShiftAcc > 
      | void FIR_MultiKernel_cincout::
      | filter(input_stream_cint16 * sin, input_cascade< cacc48, void > * cin, output_cascade< cacc48, void > * cout);
      | }
      ClassDeclTypeOptions=|
      | C[1 1]@t97@namespace SingleStream {
      | template < int NSamples, int ShiftAcc > class FIR_MultiKernel_cincout;
      | }
      ClassDecl=|
      | namespace SingleStream {
      | template < int NSamples, int ShiftAcc > class FIR_MultiKernel_cincout;
      | }
  Kernel_12 : aieBasic/AIE Class Kernel  KernelAllAttrs=|  PortNames={'sin'; 'cin'; 'cout'}  PortSerializedTypes={'{P{Tinput_stream{1{t{Scint16}}}}}'; '{P{Tinput_cascade{2{t{Scacc48}}{t{Bv}}}}}'; '{P{Toutput_cascade{2{t{Scacc48}}{t{Bv}}}}}'}  PortWindowSizes={0.000000000000000000e+00; 0.000000000000000000e+00; 0.000000000000000000e+00}  PortWindowMargins={0.000000000000000000e+00; 0.000000000000000000e+00; 0.000000000000000000e+00}  PortSynchronicities={'auto', 'auto', 'auto'}  PortSignalSizes={0.000000000000000000e+00; 0.000000000000000000e+00; 5.120000000000000000e+02}  ClassTemplateSpecKind=implicit  ClassTemplateParamNames={'NSamples'; 'ShiftAcc'}  ClassTemplateParamKinds={'nontype'; 'nontype'}  ClassTemplateParamTypes={'int'; 'int'}  ClassTemplateParamValues={'512', '15'}  ClassCtorParamNames={'taps'; 'Delay'}  ClassCtorParamSerializedTypes={'{R{Q1{C{Scint16}8}}}'; '{Q1{Bi32}}'}  ClassCtorParamValues={'[14-121i 342-439i 1454-497i 8773+2748i 237+96i 102+525i -121+233i -54+21i]', '1'}  ClassIndex=1  ClassCtorIndex=1  ClassTabVisible=on  ClassTemplateParamsVisible=on  ClassCtorDeclVisible=on  ClassCtorParamsVisible=on  FunctionTabVisible=on  FunctionDecl=|  PortAttrs={ 'input', 'sin', 'input_stream_cint16 *', '', '0', '', ''; 'input', 'cin', 'input_cascade< cacc48, void > *', '', '0', '', ''; 'output', 'cout', 'output_cascade< cacc48, void > *', '', '', '', 'N' }  PortAttrsEnables={'off', 'off', 'off', 'off', 'off', 'off', 'off';'off', 'off', 'off', 'off', 'off', 'off', 'off';'off', 'off', 'off', 'off', 'off', 'off', 'on'}  SampleTime=-1  ClassDeclTypeOptions=|  ClassDecl=|  ClassTemplateParams={ 'NSamples', 'int', 'BURST_LENGTH'; 'ShiftAcc', 'int', 'SHIFT_ACC' }  ClassTemplateParamsEnables={'off', 'off', 'on';'off', 'off', 'on'}  ClassCtorDeclTypeOptions=C[1 1]@t73@FIR_MultiKernel_cincout(cint16 const ( & taps ) [ 8 ], int32 const Delay)  ClassCtorDecl=FIR_MultiKernel_cincout(cint16 const ( & taps ) [ 8 ], int32 const Delay)  ClassCtorParams={ 'taps', 'cint16 const ( &) [ 8 ]', 'phi_3'; 'Delay', 'int32 const', '1' }  KernelHeaderFile=FirSingleStream.h  KernelClassName=SingleStream::FIR_MultiKernel_cincout  KernelFunction=filter  KernelSourceFile=FirSingleStream.cpp  KernelSearchPaths={'$SRC', '$SRC/aie_kernels'}  PreProcOptions={}  blockJsonConstraints=[]
      KernelAllAttrs=|
      | s[12;12;9;9;19;14;21;23;21;23;24;21;15;17;12;24;26;26;26;27;28;9;21;23;23;23;24;25;14;19;19;29]@FunctionNameDeclFileNamePortNamesPortTypesPortSerializedTypesPortDirectionsPortWindowSizeEnablesPortWindowMarginEnablesPortBufferSizeEnablesPortBufferMarginEnablesPortSynchronicityEnablesPortSignalSizeEnablesPortBufferSizesPortBufferMarginsFunctionDeclFunctionTemplateSpecKindFunctionTemplateParamNamesFunctionTemplateParamKindsFunctionTemplateParamTypesFunctionTemplateParamValuesFunctionTemplateParamEnablesClassDeclClassTemplateSpecKindClassTemplateParamNamesClassTemplateParamKindsClassTemplateParamTypesClassTemplateParamValuesClassTemplateParamEnablesClassCtorDeclsClassCtorParamNamesClassCtorParamTypesClassCtorParamSerializedTypes[1 1]@C[32 1]@t6@filtert39@../../src/aie_kernels/FirSingleStream.hC[3 1]@t3@sint3@cint4@coutC[3 1]@t21@input_stream_cint16 *t31@input_cascade< cacc48, void > *t32@output_cascade< cacc48, void > *C[3 1]@t33@{P{Tinput_stream{1{t{Scint16}}}}}t41@{P{Tinput_cascade{2{t{Scacc48}}{t{Bv}}}}}t42@{P{Toutput_cascade{2{t{Scacc48}}{t{Bv}}}}}C[3 1]@t5@inputt5@inputt6@outputC[3 1]@l0@l0@l0@C[3 1]@l0@l0@l0@C[3 1]@l0@l0@l0@C[3 1]@l0@l0@l0@C[3 1]@l0@l0@l0@C[3 1]@l0@l0@l1@C[3 1]@nnnC[3 1]@nnnt209@namespace SingleStream {
      | template < int NSamples, int ShiftAcc > 
      | void FIR_MultiKernel_cincout::
      | filter(input_stream_cint16 * sin, input_cascade< cacc48, void > * cin, output_cascade< cacc48, void > * cout);
      | }t4@nonee[0 1]@e[0 1]@e[0 1]@e[0 1]@e[0 1]@t97@namespace SingleStream {
      | template < int NSamples, int ShiftAcc > class FIR_MultiKernel_cincout;
      | }t8@implicitC[2 1]@t8@NSamplest8@ShiftAccC[2 1]@t7@nontypet7@nontypeC[2 1]@t3@intt3@intC[2 1]@nnC[2 1]@l1@l1@C[1 1]@t73@FIR_MultiKernel_cincout(cint16 const ( & taps ) [ 8 ], int32 const Delay)C[1 1]@C[2 1]@t4@tapst5@DelayC[1 1]@C[2 1]@t23@cint16 const ( &) [ 8 ]t11@int32 constC[1 1]@C[2 1]@t20@{R{Q1{C{Scint16}8}}}t10@{Q1{Bi32}}
      FunctionDecl=|
      | namespace SingleStream {
      | template < int NSamples, int ShiftAcc > 
      | void FIR_MultiKernel_cincout::
      | filter(input_stream_cint16 * sin, input_cascade< cacc48, void > * cin, output_cascade< cacc48, void > * cout);
      | }
      ClassDeclTypeOptions=|
      | C[1 1]@t97@namespace SingleStream {
      | template < int NSamples, int ShiftAcc > class FIR_MultiKernel_cincout;
      | }
      ClassDecl=|
      | namespace SingleStream {
      | template < int NSamples, int ShiftAcc > class FIR_MultiKernel_cincout;
      | }
  Kernel_13 : aieBasic/AIE Class Kernel  KernelAllAttrs=|  PortNames={'sin'; 'cin'; 'cout'}  PortSerializedTypes={'{P{Tinput_stream{1{t{Scint16}}}}}'; '{P{Tinput_cascade{2{t{Scacc48}}{t{Bv}}}}}'; '{P{Toutput_cascade{2{t{Scacc48}}{t{Bv}}}}}'}  PortWindowSizes={0.000000000000000000e+00; 0.000000000000000000e+00; 0.000000000000000000e+00}  PortWindowMargins={0.000000000000000000e+00; 0.000000000000000000e+00; 0.000000000000000000e+00}  PortSynchronicities={'auto', 'auto', 'auto'}  PortSignalSizes={0.000000000000000000e+00; 0.000000000000000000e+00; 5.120000000000000000e+02}  ClassTemplateSpecKind=implicit  ClassTemplateParamNames={'NSamples'; 'ShiftAcc'}  ClassTemplateParamKinds={'nontype'; 'nontype'}  ClassTemplateParamTypes={'int'; 'int'}  ClassTemplateParamValues={'512', '15'}  ClassCtorParamNames={'taps'; 'Delay'}  ClassCtorParamSerializedTypes={'{R{Q1{C{Scint16}8}}}'; '{Q1{Bi32}}'}  ClassCtorParamValues={'[-21+26i 146-91i 1183+239i 4086+5221i 248-2878i 237-54i -160+111i -83-21i]', '1'}  ClassIndex=1  ClassCtorIndex=1  ClassTabVisible=on  ClassTemplateParamsVisible=on  ClassCtorDeclVisible=on  ClassCtorParamsVisible=on  FunctionTabVisible=on  FunctionDecl=|  PortAttrs={ 'input', 'sin', 'input_stream_cint16 *', '', '0', '', ''; 'input', 'cin', 'input_cascade< cacc48, void > *', '', '0', '', ''; 'output', 'cout', 'output_cascade< cacc48, void > *', '', '', '', 'N' }  PortAttrsEnables={'off', 'off', 'off', 'off', 'off', 'off', 'off';'off', 'off', 'off', 'off', 'off', 'off', 'off';'off', 'off', 'off', 'off', 'off', 'off', 'on'}  SampleTime=-1  ClassDeclTypeOptions=|  ClassDecl=|  ClassTemplateParams={ 'NSamples', 'int', 'BURST_LENGTH'; 'ShiftAcc', 'int', 'SHIFT_ACC' }  ClassTemplateParamsEnables={'off', 'off', 'on';'off', 'off', 'on'}  ClassCtorDeclTypeOptions=C[1 1]@t73@FIR_MultiKernel_cincout(cint16 const ( & taps ) [ 8 ], int32 const Delay)  ClassCtorDecl=FIR_MultiKernel_cincout(cint16 const ( & taps ) [ 8 ], int32 const Delay)  ClassCtorParams={ 'taps', 'cint16 const ( &) [ 8 ]', 'phi_2'; 'Delay', 'int32 const', '1' }  KernelHeaderFile=FirSingleStream.h  KernelClassName=SingleStream::FIR_MultiKernel_cincout  KernelFunction=filter  KernelSourceFile=FirSingleStream.cpp  KernelSearchPaths={'$SRC', '$SRC/aie_kernels'}  PreProcOptions={}  blockJsonConstraints=[]
      KernelAllAttrs=|
      | s[12;12;9;9;19;14;21;23;21;23;24;21;15;17;12;24;26;26;26;27;28;9;21;23;23;23;24;25;14;19;19;29]@FunctionNameDeclFileNamePortNamesPortTypesPortSerializedTypesPortDirectionsPortWindowSizeEnablesPortWindowMarginEnablesPortBufferSizeEnablesPortBufferMarginEnablesPortSynchronicityEnablesPortSignalSizeEnablesPortBufferSizesPortBufferMarginsFunctionDeclFunctionTemplateSpecKindFunctionTemplateParamNamesFunctionTemplateParamKindsFunctionTemplateParamTypesFunctionTemplateParamValuesFunctionTemplateParamEnablesClassDeclClassTemplateSpecKindClassTemplateParamNamesClassTemplateParamKindsClassTemplateParamTypesClassTemplateParamValuesClassTemplateParamEnablesClassCtorDeclsClassCtorParamNamesClassCtorParamTypesClassCtorParamSerializedTypes[1 1]@C[32 1]@t6@filtert39@../../src/aie_kernels/FirSingleStream.hC[3 1]@t3@sint3@cint4@coutC[3 1]@t21@input_stream_cint16 *t31@input_cascade< cacc48, void > *t32@output_cascade< cacc48, void > *C[3 1]@t33@{P{Tinput_stream{1{t{Scint16}}}}}t41@{P{Tinput_cascade{2{t{Scacc48}}{t{Bv}}}}}t42@{P{Toutput_cascade{2{t{Scacc48}}{t{Bv}}}}}C[3 1]@t5@inputt5@inputt6@outputC[3 1]@l0@l0@l0@C[3 1]@l0@l0@l0@C[3 1]@l0@l0@l0@C[3 1]@l0@l0@l0@C[3 1]@l0@l0@l0@C[3 1]@l0@l0@l1@C[3 1]@nnnC[3 1]@nnnt209@namespace SingleStream {
      | template < int NSamples, int ShiftAcc > 
      | void FIR_MultiKernel_cincout::
      | filter(input_stream_cint16 * sin, input_cascade< cacc48, void > * cin, output_cascade< cacc48, void > * cout);
      | }t4@nonee[0 1]@e[0 1]@e[0 1]@e[0 1]@e[0 1]@t97@namespace SingleStream {
      | template < int NSamples, int ShiftAcc > class FIR_MultiKernel_cincout;
      | }t8@implicitC[2 1]@t8@NSamplest8@ShiftAccC[2 1]@t7@nontypet7@nontypeC[2 1]@t3@intt3@intC[2 1]@nnC[2 1]@l1@l1@C[1 1]@t73@FIR_MultiKernel_cincout(cint16 const ( & taps ) [ 8 ], int32 const Delay)C[1 1]@C[2 1]@t4@tapst5@DelayC[1 1]@C[2 1]@t23@cint16 const ( &) [ 8 ]t11@int32 constC[1 1]@C[2 1]@t20@{R{Q1{C{Scint16}8}}}t10@{Q1{Bi32}}
      FunctionDecl=|
      | namespace SingleStream {
      | template < int NSamples, int ShiftAcc > 
      | void FIR_MultiKernel_cincout::
      | filter(input_stream_cint16 * sin, input_cascade< cacc48, void > * cin, output_cascade< cacc48, void > * cout);
      | }
      ClassDeclTypeOptions=|
      | C[1 1]@t97@namespace SingleStream {
      | template < int NSamples, int ShiftAcc > class FIR_MultiKernel_cincout;
      | }
      ClassDecl=|
      | namespace SingleStream {
      | template < int NSamples, int ShiftAcc > class FIR_MultiKernel_cincout;
      | }
  Kernel_20 : aieBasic/AIE Class Kernel  KernelAllAttrs=|  PortNames={'sin'; 'cin'; 'cout'}  PortSerializedTypes={'{P{Tinput_stream{1{t{Scint16}}}}}'; '{P{Tinput_cascade{2{t{Scacc48}}{t{Bv}}}}}'; '{P{Toutput_cascade{2{t{Scacc48}}{t{Bv}}}}}'}  PortWindowSizes={0.000000000000000000e+00; 0.000000000000000000e+00; 0.000000000000000000e+00}  PortWindowMargins={0.000000000000000000e+00; 0.000000000000000000e+00; 0.000000000000000000e+00}  PortSynchronicities={'auto', 'auto', 'auto'}  PortSignalSizes={0.000000000000000000e+00; 0.000000000000000000e+00; 5.120000000000000000e+02}  ClassTemplateSpecKind=implicit  ClassTemplateParamNames={'NSamples'; 'ShiftAcc'}  ClassTemplateParamKinds={'nontype'; 'nontype'}  ClassTemplateParamTypes={'int'; 'int'}  ClassTemplateParamValues={'512', '15'}  ClassCtorParamNames={'taps'; 'Delay'}  ClassCtorParamSerializedTypes={'{R{Q1{C{Scint16}8}}}'; '{Q1{Bi32}}'}  ClassCtorParamValues={'[-21+26i 146-91i 1183+239i 4086+5221i 248-2878i 237-54i -160+111i -83-21i]', '0'}  ClassIndex=1  ClassCtorIndex=1  ClassTabVisible=on  ClassTemplateParamsVisible=on  ClassCtorDeclVisible=on  ClassCtorParamsVisible=on  FunctionTabVisible=on  FunctionDecl=|  PortAttrs={ 'input', 'sin', 'input_stream_cint16 *', '', '0', '', ''; 'input', 'cin', 'input_cascade< cacc48, void > *', '', '0', '', ''; 'output', 'cout', 'output_cascade< cacc48, void > *', '', '', '', 'N' }  PortAttrsEnables={'off', 'off', 'off', 'off', 'off', 'off', 'off';'off', 'off', 'off', 'off', 'off', 'off', 'off';'off', 'off', 'off', 'off', 'off', 'off', 'on'}  SampleTime=-1  ClassDeclTypeOptions=|  ClassDecl=|  ClassTemplateParams={ 'NSamples', 'int', 'BURST_LENGTH'; 'ShiftAcc', 'int', 'SHIFT_ACC' }  ClassTemplateParamsEnables={'off', 'off', 'on';'off', 'off', 'on'}  ClassCtorDeclTypeOptions=C[1 1]@t73@FIR_MultiKernel_cincout(cint16 const ( & taps ) [ 8 ], int32 const Delay)  ClassCtorDecl=FIR_MultiKernel_cincout(cint16 const ( & taps ) [ 8 ], int32 const Delay)  ClassCtorParams={ 'taps', 'cint16 const ( &) [ 8 ]', 'phi_2'; 'Delay', 'int32 const', '0' }  KernelHeaderFile=FirSingleStream.h  KernelClassName=SingleStream::FIR_MultiKernel_cincout  KernelFunction=filter  KernelSourceFile=FirSingleStream.cpp  KernelSearchPaths={'$SRC', '$SRC/aie_kernels'}  PreProcOptions={}  blockJsonConstraints=[]
      KernelAllAttrs=|
      | s[12;12;9;9;19;14;21;23;21;23;24;21;15;17;12;24;26;26;26;27;28;9;21;23;23;23;24;25;14;19;19;29]@FunctionNameDeclFileNamePortNamesPortTypesPortSerializedTypesPortDirectionsPortWindowSizeEnablesPortWindowMarginEnablesPortBufferSizeEnablesPortBufferMarginEnablesPortSynchronicityEnablesPortSignalSizeEnablesPortBufferSizesPortBufferMarginsFunctionDeclFunctionTemplateSpecKindFunctionTemplateParamNamesFunctionTemplateParamKindsFunctionTemplateParamTypesFunctionTemplateParamValuesFunctionTemplateParamEnablesClassDeclClassTemplateSpecKindClassTemplateParamNamesClassTemplateParamKindsClassTemplateParamTypesClassTemplateParamValuesClassTemplateParamEnablesClassCtorDeclsClassCtorParamNamesClassCtorParamTypesClassCtorParamSerializedTypes[1 1]@C[32 1]@t6@filtert39@../../src/aie_kernels/FirSingleStream.hC[3 1]@t3@sint3@cint4@coutC[3 1]@t21@input_stream_cint16 *t31@input_cascade< cacc48, void > *t32@output_cascade< cacc48, void > *C[3 1]@t33@{P{Tinput_stream{1{t{Scint16}}}}}t41@{P{Tinput_cascade{2{t{Scacc48}}{t{Bv}}}}}t42@{P{Toutput_cascade{2{t{Scacc48}}{t{Bv}}}}}C[3 1]@t5@inputt5@inputt6@outputC[3 1]@l0@l0@l0@C[3 1]@l0@l0@l0@C[3 1]@l0@l0@l0@C[3 1]@l0@l0@l0@C[3 1]@l0@l0@l0@C[3 1]@l0@l0@l1@C[3 1]@nnnC[3 1]@nnnt209@namespace SingleStream {
      | template < int NSamples, int ShiftAcc > 
      | void FIR_MultiKernel_cincout::
      | filter(input_stream_cint16 * sin, input_cascade< cacc48, void > * cin, output_cascade< cacc48, void > * cout);
      | }t4@nonee[0 1]@e[0 1]@e[0 1]@e[0 1]@e[0 1]@t97@namespace SingleStream {
      | template < int NSamples, int ShiftAcc > class FIR_MultiKernel_cincout;
      | }t8@implicitC[2 1]@t8@NSamplest8@ShiftAccC[2 1]@t7@nontypet7@nontypeC[2 1]@t3@intt3@intC[2 1]@nnC[2 1]@l1@l1@C[1 1]@t73@FIR_MultiKernel_cincout(cint16 const ( & taps ) [ 8 ], int32 const Delay)C[1 1]@C[2 1]@t4@tapst5@DelayC[1 1]@C[2 1]@t23@cint16 const ( &) [ 8 ]t11@int32 constC[1 1]@C[2 1]@t20@{R{Q1{C{Scint16}8}}}t10@{Q1{Bi32}}
      FunctionDecl=|
      | namespace SingleStream {
      | template < int NSamples, int ShiftAcc > 
      | void FIR_MultiKernel_cincout::
      | filter(input_stream_cint16 * sin, input_cascade< cacc48, void > * cin, output_cascade< cacc48, void > * cout);
      | }
      ClassDeclTypeOptions=|
      | C[1 1]@t97@namespace SingleStream {
      | template < int NSamples, int ShiftAcc > class FIR_MultiKernel_cincout;
      | }
      ClassDecl=|
      | namespace SingleStream {
      | template < int NSamples, int ShiftAcc > class FIR_MultiKernel_cincout;
      | }
  Kernel_21 : aieBasic/AIE Class Kernel  KernelAllAttrs=|  PortNames={'sin'; 'cin'; 'cout'}  PortSerializedTypes={'{P{Tinput_stream{1{t{Scint16}}}}}'; '{P{Tinput_cascade{2{t{Scacc48}}{t{Bv}}}}}'; '{P{Toutput_cascade{2{t{Scacc48}}{t{Bv}}}}}'}  PortWindowSizes={0.000000000000000000e+00; 0.000000000000000000e+00; 0.000000000000000000e+00}  PortWindowMargins={0.000000000000000000e+00; 0.000000000000000000e+00; 0.000000000000000000e+00}  PortSynchronicities={'auto', 'auto', 'auto'}  PortSignalSizes={0.000000000000000000e+00; 0.000000000000000000e+00; 5.120000000000000000e+02}  ClassTemplateSpecKind=implicit  ClassTemplateParamNames={'NSamples'; 'ShiftAcc'}  ClassTemplateParamKinds={'nontype'; 'nontype'}  ClassTemplateParamTypes={'int'; 'int'}  ClassTemplateParamValues={'512', '15'}  ClassCtorParamNames={'taps'; 'Delay'}  ClassCtorParamSerializedTypes={'{R{Q1{C{Scint16}8}}}'; '{Q1{Bi32}}'}  ClassCtorParamValues={'[-83+21i -160-111i 237+54i 248+2878i 4086-5221i 1183-239i 146+91i -21-26i]', '0'}  ClassIndex=1  ClassCtorIndex=1  ClassTabVisible=on  ClassTemplateParamsVisible=on  ClassCtorDeclVisible=on  ClassCtorParamsVisible=on  FunctionTabVisible=on  FunctionDecl=|  PortAttrs={ 'input', 'sin', 'input_stream_cint16 *', '', '0', '', ''; 'input', 'cin', 'input_cascade< cacc48, void > *', '', '0', '', ''; 'output', 'cout', 'output_cascade< cacc48, void > *', '', '', '', 'N' }  PortAttrsEnables={'off', 'off', 'off', 'off', 'off', 'off', 'off';'off', 'off', 'off', 'off', 'off', 'off', 'off';'off', 'off', 'off', 'off', 'off', 'off', 'on'}  SampleTime=-1  ClassDeclTypeOptions=|  ClassDecl=|  ClassTemplateParams={ 'NSamples', 'int', 'BURST_LENGTH'; 'ShiftAcc', 'int', 'SHIFT_ACC' }  ClassTemplateParamsEnables={'off', 'off', 'on';'off', 'off', 'on'}  ClassCtorDeclTypeOptions=C[1 1]@t73@FIR_MultiKernel_cincout(cint16 const ( & taps ) [ 8 ], int32 const Delay)  ClassCtorDecl=FIR_MultiKernel_cincout(cint16 const ( & taps ) [ 8 ], int32 const Delay)  ClassCtorParams={ 'taps', 'cint16 const ( &) [ 8 ]', 'phi_1'; 'Delay', 'int32 const', '0' }  KernelHeaderFile=FirSingleStream.h  KernelClassName=SingleStream::FIR_MultiKernel_cincout  KernelFunction=filter  KernelSourceFile=FirSingleStream.cpp  KernelSearchPaths={'$SRC', '$SRC/aie_kernels'}  PreProcOptions={}  blockJsonConstraints=[]
      KernelAllAttrs=|
      | s[12;12;9;9;19;14;21;23;21;23;24;21;15;17;12;24;26;26;26;27;28;9;21;23;23;23;24;25;14;19;19;29]@FunctionNameDeclFileNamePortNamesPortTypesPortSerializedTypesPortDirectionsPortWindowSizeEnablesPortWindowMarginEnablesPortBufferSizeEnablesPortBufferMarginEnablesPortSynchronicityEnablesPortSignalSizeEnablesPortBufferSizesPortBufferMarginsFunctionDeclFunctionTemplateSpecKindFunctionTemplateParamNamesFunctionTemplateParamKindsFunctionTemplateParamTypesFunctionTemplateParamValuesFunctionTemplateParamEnablesClassDeclClassTemplateSpecKindClassTemplateParamNamesClassTemplateParamKindsClassTemplateParamTypesClassTemplateParamValuesClassTemplateParamEnablesClassCtorDeclsClassCtorParamNamesClassCtorParamTypesClassCtorParamSerializedTypes[1 1]@C[32 1]@t6@filtert39@../../src/aie_kernels/FirSingleStream.hC[3 1]@t3@sint3@cint4@coutC[3 1]@t21@input_stream_cint16 *t31@input_cascade< cacc48, void > *t32@output_cascade< cacc48, void > *C[3 1]@t33@{P{Tinput_stream{1{t{Scint16}}}}}t41@{P{Tinput_cascade{2{t{Scacc48}}{t{Bv}}}}}t42@{P{Toutput_cascade{2{t{Scacc48}}{t{Bv}}}}}C[3 1]@t5@inputt5@inputt6@outputC[3 1]@l0@l0@l0@C[3 1]@l0@l0@l0@C[3 1]@l0@l0@l0@C[3 1]@l0@l0@l0@C[3 1]@l0@l0@l0@C[3 1]@l0@l0@l1@C[3 1]@nnnC[3 1]@nnnt209@namespace SingleStream {
      | template < int NSamples, int ShiftAcc > 
      | void FIR_MultiKernel_cincout::
      | filter(input_stream_cint16 * sin, input_cascade< cacc48, void > * cin, output_cascade< cacc48, void > * cout);
      | }t4@nonee[0 1]@e[0 1]@e[0 1]@e[0 1]@e[0 1]@t97@namespace SingleStream {
      | template < int NSamples, int ShiftAcc > class FIR_MultiKernel_cincout;
      | }t8@implicitC[2 1]@t8@NSamplest8@ShiftAccC[2 1]@t7@nontypet7@nontypeC[2 1]@t3@intt3@intC[2 1]@nnC[2 1]@l1@l1@C[1 1]@t73@FIR_MultiKernel_cincout(cint16 const ( & taps ) [ 8 ], int32 const Delay)C[1 1]@C[2 1]@t4@tapst5@DelayC[1 1]@C[2 1]@t23@cint16 const ( &) [ 8 ]t11@int32 constC[1 1]@C[2 1]@t20@{R{Q1{C{Scint16}8}}}t10@{Q1{Bi32}}
      FunctionDecl=|
      | namespace SingleStream {
      | template < int NSamples, int ShiftAcc > 
      | void FIR_MultiKernel_cincout::
      | filter(input_stream_cint16 * sin, input_cascade< cacc48, void > * cin, output_cascade< cacc48, void > * cout);
      | }
      ClassDeclTypeOptions=|
      | C[1 1]@t97@namespace SingleStream {
      | template < int NSamples, int ShiftAcc > class FIR_MultiKernel_cincout;
      | }
      ClassDecl=|
      | namespace SingleStream {
      | template < int NSamples, int ShiftAcc > class FIR_MultiKernel_cincout;
      | }
  Kernel_22 : aieBasic/AIE Class Kernel  KernelAllAttrs=|  PortNames={'sin'; 'cin'; 'cout'}  PortSerializedTypes={'{P{Tinput_stream{1{t{Scint16}}}}}'; '{P{Tinput_cascade{2{t{Scacc48}}{t{Bv}}}}}'; '{P{Toutput_cascade{2{t{Scacc48}}{t{Bv}}}}}'}  PortWindowSizes={0.000000000000000000e+00; 0.000000000000000000e+00; 0.000000000000000000e+00}  PortWindowMargins={0.000000000000000000e+00; 0.000000000000000000e+00; 0.000000000000000000e+00}  PortSynchronicities={'auto', 'auto', 'auto'}  PortSignalSizes={0.000000000000000000e+00; 0.000000000000000000e+00; 5.120000000000000000e+02}  ClassTemplateSpecKind=implicit  ClassTemplateParamNames={'NSamples'; 'ShiftAcc'}  ClassTemplateParamKinds={'nontype'; 'nontype'}  ClassTemplateParamTypes={'int'; 'int'}  ClassTemplateParamValues={'512', '15'}  ClassCtorParamNames={'taps'; 'Delay'}  ClassCtorParamSerializedTypes={'{R{Q1{C{Scint16}8}}}'; '{Q1{Bi32}}'}  ClassCtorParamValues={'[-54-21i -121-233i 102-525i 237-96i 8773-2748i 1454+497i 342+439i 14+121i]', '0'}  ClassIndex=1  ClassCtorIndex=1  ClassTabVisible=on  ClassTemplateParamsVisible=on  ClassCtorDeclVisible=on  ClassCtorParamsVisible=on  FunctionTabVisible=on  FunctionDecl=|  PortAttrs={ 'input', 'sin', 'input_stream_cint16 *', '', '0', '', ''; 'input', 'cin', 'input_cascade< cacc48, void > *', '', '0', '', ''; 'output', 'cout', 'output_cascade< cacc48, void > *', '', '', '', 'N' }  PortAttrsEnables={'off', 'off', 'off', 'off', 'off', 'off', 'off';'off', 'off', 'off', 'off', 'off', 'off', 'off';'off', 'off', 'off', 'off', 'off', 'off', 'on'}  SampleTime=-1  ClassDeclTypeOptions=|  ClassDecl=|  ClassTemplateParams={ 'NSamples', 'int', 'BURST_LENGTH'; 'ShiftAcc', 'int', 'SHIFT_ACC' }  ClassTemplateParamsEnables={'off', 'off', 'on';'off', 'off', 'on'}  ClassCtorDeclTypeOptions=C[1 1]@t73@FIR_MultiKernel_cincout(cint16 const ( & taps ) [ 8 ], int32 const Delay)  ClassCtorDecl=FIR_MultiKernel_cincout(cint16 const ( & taps ) [ 8 ], int32 const Delay)  ClassCtorParams={ 'taps', 'cint16 const ( &) [ 8 ]', 'phi_0'; 'Delay', 'int32 const', '0' }  KernelHeaderFile=FirSingleStream.h  KernelClassName=SingleStream::FIR_MultiKernel_cincout  KernelFunction=filter  KernelSourceFile=FirSingleStream.cpp  KernelSearchPaths={'$SRC', '$SRC/aie_kernels'}  PreProcOptions={}  blockJsonConstraints=[]
      KernelAllAttrs=|
      | s[12;12;9;9;19;14;21;23;21;23;24;21;15;17;12;24;26;26;26;27;28;9;21;23;23;23;24;25;14;19;19;29]@FunctionNameDeclFileNamePortNamesPortTypesPortSerializedTypesPortDirectionsPortWindowSizeEnablesPortWindowMarginEnablesPortBufferSizeEnablesPortBufferMarginEnablesPortSynchronicityEnablesPortSignalSizeEnablesPortBufferSizesPortBufferMarginsFunctionDeclFunctionTemplateSpecKindFunctionTemplateParamNamesFunctionTemplateParamKindsFunctionTemplateParamTypesFunctionTemplateParamValuesFunctionTemplateParamEnablesClassDeclClassTemplateSpecKindClassTemplateParamNamesClassTemplateParamKindsClassTemplateParamTypesClassTemplateParamValuesClassTemplateParamEnablesClassCtorDeclsClassCtorParamNamesClassCtorParamTypesClassCtorParamSerializedTypes[1 1]@C[32 1]@t6@filtert39@../../src/aie_kernels/FirSingleStream.hC[3 1]@t3@sint3@cint4@coutC[3 1]@t21@input_stream_cint16 *t31@input_cascade< cacc48, void > *t32@output_cascade< cacc48, void > *C[3 1]@t33@{P{Tinput_stream{1{t{Scint16}}}}}t41@{P{Tinput_cascade{2{t{Scacc48}}{t{Bv}}}}}t42@{P{Toutput_cascade{2{t{Scacc48}}{t{Bv}}}}}C[3 1]@t5@inputt5@inputt6@outputC[3 1]@l0@l0@l0@C[3 1]@l0@l0@l0@C[3 1]@l0@l0@l0@C[3 1]@l0@l0@l0@C[3 1]@l0@l0@l0@C[3 1]@l0@l0@l1@C[3 1]@nnnC[3 1]@nnnt209@namespace SingleStream {
      | template < int NSamples, int ShiftAcc > 
      | void FIR_MultiKernel_cincout::
      | filter(input_stream_cint16 * sin, input_cascade< cacc48, void > * cin, output_cascade< cacc48, void > * cout);
      | }t4@nonee[0 1]@e[0 1]@e[0 1]@e[0 1]@e[0 1]@t97@namespace SingleStream {
      | template < int NSamples, int ShiftAcc > class FIR_MultiKernel_cincout;
      | }t8@implicitC[2 1]@t8@NSamplest8@ShiftAccC[2 1]@t7@nontypet7@nontypeC[2 1]@t3@intt3@intC[2 1]@nnC[2 1]@l1@l1@C[1 1]@t73@FIR_MultiKernel_cincout(cint16 const ( & taps ) [ 8 ], int32 const Delay)C[1 1]@C[2 1]@t4@tapst5@DelayC[1 1]@C[2 1]@t23@cint16 const ( &) [ 8 ]t11@int32 constC[1 1]@C[2 1]@t20@{R{Q1{C{Scint16}8}}}t10@{Q1{Bi32}}
      FunctionDecl=|
      | namespace SingleStream {
      | template < int NSamples, int ShiftAcc > 
      | void FIR_MultiKernel_cincout::
      | filter(input_stream_cint16 * sin, input_cascade< cacc48, void > * cin, output_cascade< cacc48, void > * cout);
      | }
      ClassDeclTypeOptions=|
      | C[1 1]@t97@namespace SingleStream {
      | template < int NSamples, int ShiftAcc > class FIR_MultiKernel_cincout;
      | }
      ClassDecl=|
      | namespace SingleStream {
      | template < int NSamples, int ShiftAcc > class FIR_MultiKernel_cincout;
      | }
  Kernel_23 : aieBasic/AIE Class Kernel  KernelAllAttrs=|  PortNames={'sin'; 'cin'; 'cout'}  PortSerializedTypes={'{P{Tinput_stream{1{t{Scint16}}}}}'; '{P{Tinput_cascade{2{t{Scacc48}}{t{Bv}}}}}'; '{P{Toutput_cascade{2{t{Scacc48}}{t{Bv}}}}}'}  PortWindowSizes={0.000000000000000000e+00; 0.000000000000000000e+00; 0.000000000000000000e+00}  PortWindowMargins={0.000000000000000000e+00; 0.000000000000000000e+00; 0.000000000000000000e+00}  PortSynchronicities={'auto', 'auto', 'auto'}  PortSignalSizes={0.000000000000000000e+00; 0.000000000000000000e+00; 5.120000000000000000e+02}  ClassTemplateSpecKind=implicit  ClassTemplateParamNames={'NSamples'; 'ShiftAcc'}  ClassTemplateParamKinds={'nontype'; 'nontype'}  ClassTemplateParamTypes={'int'; 'int'}  ClassTemplateParamValues={'512', '15'}  ClassCtorParamNames={'taps'; 'Delay'}  ClassCtorParamSerializedTypes={'{R{Q1{C{Scint16}8}}}'; '{Q1{Bi32}}'}  ClassCtorParamValues={'[14-121i 342-439i 1454-497i 8773+2748i 237+96i 102+525i -121+233i -54+21i]', '1'}  ClassIndex=1  ClassCtorIndex=1  ClassTabVisible=on  ClassTemplateParamsVisible=on  ClassCtorDeclVisible=on  ClassCtorParamsVisible=on  FunctionTabVisible=on  FunctionDecl=|  PortAttrs={ 'input', 'sin', 'input_stream_cint16 *', '', '0', '', ''; 'input', 'cin', 'input_cascade< cacc48, void > *', '', '0', '', ''; 'output', 'cout', 'output_cascade< cacc48, void > *', '', '', '', 'N' }  PortAttrsEnables={'off', 'off', 'off', 'off', 'off', 'off', 'off';'off', 'off', 'off', 'off', 'off', 'off', 'off';'off', 'off', 'off', 'off', 'off', 'off', 'on'}  SampleTime=-1  ClassDeclTypeOptions=|  ClassDecl=|  ClassTemplateParams={ 'NSamples', 'int', 'BURST_LENGTH'; 'ShiftAcc', 'int', 'SHIFT_ACC' }  ClassTemplateParamsEnables={'off', 'off', 'on';'off', 'off', 'on'}  ClassCtorDeclTypeOptions=C[1 1]@t73@FIR_MultiKernel_cincout(cint16 const ( & taps ) [ 8 ], int32 const Delay)  ClassCtorDecl=FIR_MultiKernel_cincout(cint16 const ( & taps ) [ 8 ], int32 const Delay)  ClassCtorParams={ 'taps', 'cint16 const ( &) [ 8 ]', 'phi_3'; 'Delay', 'int32 const', '1' }  KernelHeaderFile=FirSingleStream.h  KernelClassName=SingleStream::FIR_MultiKernel_cincout  KernelFunction=filter  KernelSourceFile=FirSingleStream.cpp  KernelSearchPaths={'$SRC', '$SRC/aie_kernels'}  PreProcOptions={}  blockJsonConstraints=[]
      KernelAllAttrs=|
      | s[12;12;9;9;19;14;21;23;21;23;24;21;15;17;12;24;26;26;26;27;28;9;21;23;23;23;24;25;14;19;19;29]@FunctionNameDeclFileNamePortNamesPortTypesPortSerializedTypesPortDirectionsPortWindowSizeEnablesPortWindowMarginEnablesPortBufferSizeEnablesPortBufferMarginEnablesPortSynchronicityEnablesPortSignalSizeEnablesPortBufferSizesPortBufferMarginsFunctionDeclFunctionTemplateSpecKindFunctionTemplateParamNamesFunctionTemplateParamKindsFunctionTemplateParamTypesFunctionTemplateParamValuesFunctionTemplateParamEnablesClassDeclClassTemplateSpecKindClassTemplateParamNamesClassTemplateParamKindsClassTemplateParamTypesClassTemplateParamValuesClassTemplateParamEnablesClassCtorDeclsClassCtorParamNamesClassCtorParamTypesClassCtorParamSerializedTypes[1 1]@C[32 1]@t6@filtert39@../../src/aie_kernels/FirSingleStream.hC[3 1]@t3@sint3@cint4@coutC[3 1]@t21@input_stream_cint16 *t31@input_cascade< cacc48, void > *t32@output_cascade< cacc48, void > *C[3 1]@t33@{P{Tinput_stream{1{t{Scint16}}}}}t41@{P{Tinput_cascade{2{t{Scacc48}}{t{Bv}}}}}t42@{P{Toutput_cascade{2{t{Scacc48}}{t{Bv}}}}}C[3 1]@t5@inputt5@inputt6@outputC[3 1]@l0@l0@l0@C[3 1]@l0@l0@l0@C[3 1]@l0@l0@l0@C[3 1]@l0@l0@l0@C[3 1]@l0@l0@l0@C[3 1]@l0@l0@l1@C[3 1]@nnnC[3 1]@nnnt209@namespace SingleStream {
      | template < int NSamples, int ShiftAcc > 
      | void FIR_MultiKernel_cincout::
      | filter(input_stream_cint16 * sin, input_cascade< cacc48, void > * cin, output_cascade< cacc48, void > * cout);
      | }t4@nonee[0 1]@e[0 1]@e[0 1]@e[0 1]@e[0 1]@t97@namespace SingleStream {
      | template < int NSamples, int ShiftAcc > class FIR_MultiKernel_cincout;
      | }t8@implicitC[2 1]@t8@NSamplest8@ShiftAccC[2 1]@t7@nontypet7@nontypeC[2 1]@t3@intt3@intC[2 1]@nnC[2 1]@l1@l1@C[1 1]@t73@FIR_MultiKernel_cincout(cint16 const ( & taps ) [ 8 ], int32 const Delay)C[1 1]@C[2 1]@t4@tapst5@DelayC[1 1]@C[2 1]@t23@cint16 const ( &) [ 8 ]t11@int32 constC[1 1]@C[2 1]@t20@{R{Q1{C{Scint16}8}}}t10@{Q1{Bi32}}
      FunctionDecl=|
      | namespace SingleStream {
      | template < int NSamples, int ShiftAcc > 
      | void FIR_MultiKernel_cincout::
      | filter(input_stream_cint16 * sin, input_cascade< cacc48, void > * cin, output_cascade< cacc48, void > * cout);
      | }
      ClassDeclTypeOptions=|
      | C[1 1]@t97@namespace SingleStream {
      | template < int NSamples, int ShiftAcc > class FIR_MultiKernel_cincout;
      | }
      ClassDecl=|
      | namespace SingleStream {
      | template < int NSamples, int ShiftAcc > class FIR_MultiKernel_cincout;
      | }
  Kernel_30 : aieBasic/AIE Class Kernel  KernelAllAttrs=|  PortNames={'sin'; 'cin'; 'sout'}  PortSerializedTypes={'{P{Tinput_stream{1{t{Scint16}}}}}'; '{P{Tinput_cascade{2{t{Scacc48}}{t{Bv}}}}}'; '{P{Toutput_stream{1{t{Scint16}}}}}'}  PortWindowSizes={0.000000000000000000e+00; 0.000000000000000000e+00; 0.000000000000000000e+00}  PortWindowMargins={0.000000000000000000e+00; 0.000000000000000000e+00; 0.000000000000000000e+00}  PortSynchronicities={'auto', 'auto', 'auto'}  PortSignalSizes={0.000000000000000000e+00; 0.000000000000000000e+00; 5.120000000000000000e+02}  ClassTemplateSpecKind=implicit  ClassTemplateParamNames={'NSamples'; 'ShiftAcc'}  ClassTemplateParamKinds={'nontype'; 'nontype'}  ClassTemplateParamTypes={'int'; 'int'}  ClassTemplateParamValues={'512', '15'}  ClassCtorParamNames={'taps'; 'Delay'}  ClassCtorParamSerializedTypes={'{R{Q1{C{Scint16}8}}}'; '{Q1{Bi32}}'}  ClassCtorParamValues={'[14-121i 342-439i 1454-497i 8773+2748i 237+96i 102+525i -121+233i -54+21i]', '0'}  ClassIndex=1  ClassCtorIndex=1  ClassTabVisible=on  ClassTemplateParamsVisible=on  ClassCtorDeclVisible=on  ClassCtorParamsVisible=on  FunctionTabVisible=on  FunctionDecl=|  PortAttrs={ 'input', 'sin', 'input_stream_cint16 *', '', '0', '', ''; 'input', 'cin', 'input_cascade< cacc48, void > *', '', '0', '', ''; 'output', 'sout', 'output_stream_cint16 *', '', '', '', 'N' }  PortAttrsEnables={'off', 'off', 'off', 'off', 'off', 'off', 'off';'off', 'off', 'off', 'off', 'off', 'off', 'off';'off', 'off', 'off', 'off', 'off', 'off', 'on'}  SampleTime=-1  ClassDeclTypeOptions=|  ClassDecl=|  ClassTemplateParams={ 'NSamples', 'int', 'BURST_LENGTH'; 'ShiftAcc', 'int', 'SHIFT_ACC' }  ClassTemplateParamsEnables={'off', 'off', 'on';'off', 'off', 'on'}  ClassCtorDeclTypeOptions=C[1 1]@t69@FIR_MultiKernel_cin(cint16 const ( & taps ) [ 8 ], int32 const Delay)  ClassCtorDecl=FIR_MultiKernel_cin(cint16 const ( & taps ) [ 8 ], int32 const Delay)  ClassCtorParams={ 'taps', 'cint16 const ( &) [ 8 ]', 'phi_3'; 'Delay', 'int32 const', '0' }  KernelHeaderFile=FirSingleStream.h  KernelClassName=SingleStream::FIR_MultiKernel_cin  KernelFunction=filter  KernelSourceFile=FirSingleStream.cpp  KernelSearchPaths={'$SRC', '$SRC/aie_kernels'}  PreProcOptions={}  blockJsonConstraints=[]
      KernelAllAttrs=|
      | s[12;12;9;9;19;14;21;23;21;23;24;21;15;17;12;24;26;26;26;27;28;9;21;23;23;23;24;25;14;19;19;29]@FunctionNameDeclFileNamePortNamesPortTypesPortSerializedTypesPortDirectionsPortWindowSizeEnablesPortWindowMarginEnablesPortBufferSizeEnablesPortBufferMarginEnablesPortSynchronicityEnablesPortSignalSizeEnablesPortBufferSizesPortBufferMarginsFunctionDeclFunctionTemplateSpecKindFunctionTemplateParamNamesFunctionTemplateParamKindsFunctionTemplateParamTypesFunctionTemplateParamValuesFunctionTemplateParamEnablesClassDeclClassTemplateSpecKindClassTemplateParamNamesClassTemplateParamKindsClassTemplateParamTypesClassTemplateParamValuesClassTemplateParamEnablesClassCtorDeclsClassCtorParamNamesClassCtorParamTypesClassCtorParamSerializedTypes[1 1]@C[32 1]@t6@filtert39@../../src/aie_kernels/FirSingleStream.hC[3 1]@t3@sint3@cint4@soutC[3 1]@t21@input_stream_cint16 *t31@input_cascade< cacc48, void > *t22@output_stream_cint16 *C[3 1]@t33@{P{Tinput_stream{1{t{Scint16}}}}}t41@{P{Tinput_cascade{2{t{Scacc48}}{t{Bv}}}}}t34@{P{Toutput_stream{1{t{Scint16}}}}}C[3 1]@t5@inputt5@inputt6@outputC[3 1]@l0@l0@l0@C[3 1]@l0@l0@l0@C[3 1]@l0@l0@l0@C[3 1]@l0@l0@l0@C[3 1]@l0@l0@l0@C[3 1]@l0@l0@l1@C[3 1]@nnnC[3 1]@nnnt195@namespace SingleStream {
      | template < int NSamples, int ShiftAcc > 
      | void FIR_MultiKernel_cin::
      | filter(input_stream_cint16 * sin, input_cascade< cacc48, void > * cin, output_stream_cint16 * sout);
      | }t4@nonee[0 1]@e[0 1]@e[0 1]@e[0 1]@e[0 1]@t93@namespace SingleStream {
      | template < int NSamples, int ShiftAcc > class FIR_MultiKernel_cin;
      | }t8@implicitC[2 1]@t8@NSamplest8@ShiftAccC[2 1]@t7@nontypet7@nontypeC[2 1]@t3@intt3@intC[2 1]@nnC[2 1]@l1@l1@C[1 1]@t69@FIR_MultiKernel_cin(cint16 const ( & taps ) [ 8 ], int32 const Delay)C[1 1]@C[2 1]@t4@tapst5@DelayC[1 1]@C[2 1]@t23@cint16 const ( &) [ 8 ]t11@int32 constC[1 1]@C[2 1]@t20@{R{Q1{C{Scint16}8}}}t10@{Q1{Bi32}}
      FunctionDecl=|
      | namespace SingleStream {
      | template < int NSamples, int ShiftAcc > 
      | void FIR_MultiKernel_cin::
      | filter(input_stream_cint16 * sin, input_cascade< cacc48, void > * cin, output_stream_cint16 * sout);
      | }
      ClassDeclTypeOptions=|
      | C[1 1]@t93@namespace SingleStream {
      | template < int NSamples, int ShiftAcc > class FIR_MultiKernel_cin;
      | }
      ClassDecl=|
      | namespace SingleStream {
      | template < int NSamples, int ShiftAcc > class FIR_MultiKernel_cin;
      | }
  Kernel_31 : aieBasic/AIE Class Kernel  KernelAllAttrs=|  PortNames={'sin'; 'cout'}  PortSerializedTypes={'{P{Tinput_stream{1{t{Scint16}}}}}'; '{P{Toutput_cascade{2{t{Scacc48}}{t{Bv}}}}}'}  PortWindowSizes={0.000000000000000000e+00; 0.000000000000000000e+00}  PortWindowMargins={0.000000000000000000e+00; 0.000000000000000000e+00}  PortSynchronicities={'auto', 'auto'}  PortSignalSizes={0.000000000000000000e+00; 5.120000000000000000e+02}  ClassTemplateSpecKind=implicit  ClassTemplateParamNames={'NSamples'; 'ShiftAcc'}  ClassTemplateParamKinds={'nontype'; 'nontype'}  ClassTemplateParamTypes={'int'; 'int'}  ClassTemplateParamValues={'512', '15'}  ClassCtorParamNames={'taps'; 'Delay'}  ClassCtorParamSerializedTypes={'{R{Q1{C{Scint16}8}}}'; '{Q1{Bi32}}'}  ClassCtorParamValues={'[-21+26i 146-91i 1183+239i 4086+5221i 248-2878i 237-54i -160+111i -83-21i]', '0'}  ClassIndex=1  ClassCtorIndex=1  ClassTabVisible=on  ClassTemplateParamsVisible=on  ClassCtorDeclVisible=on  ClassCtorParamsVisible=on  FunctionTabVisible=on  FunctionDecl=|  PortAttrs={ 'input', 'sin', 'input_stream_cint16 *', '', '0', '', ''; 'output', 'cout', 'output_cascade< cacc48, void > *', '', '', '', 'N' }  PortAttrsEnables={'off', 'off', 'off', 'off', 'off', 'off', 'off';'off', 'off', 'off', 'off', 'off', 'off', 'on'}  SampleTime=-1  ClassDeclTypeOptions=|  ClassDecl=|  ClassTemplateParams={ 'NSamples', 'int', 'BURST_LENGTH'; 'ShiftAcc', 'int', 'SHIFT_ACC' }  ClassTemplateParamsEnables={'off', 'off', 'on';'off', 'off', 'on'}  ClassCtorDeclTypeOptions=C[1 1]@t70@FIR_MultiKernel_cout(cint16 const ( & taps ) [ 8 ], int32 const Delay)  ClassCtorDecl=FIR_MultiKernel_cout(cint16 const ( & taps ) [ 8 ], int32 const Delay)  ClassCtorParams={ 'taps', 'cint16 const ( &) [ 8 ]', 'phi_2'; 'Delay', 'int32 const', '0' }  KernelHeaderFile=FirSingleStream.h  KernelClassName=SingleStream::FIR_MultiKernel_cout  KernelFunction=filter  KernelSourceFile=FirSingleStream.cpp  KernelSearchPaths={'$SRC', '$SRC/aie_kernels'}  PreProcOptions={}  blockJsonConstraints="{\"type\":\"constraint\",\"constraintType\":\"location_kernel\",\"sid\":\"388\",\"lhs\":{\"type\":\"location\",\"templParam\":\"kernel\",\"args\":{\"type\":\"kernel\",\"name\":\"SingleStreamSSR/SSR4/Kernel_31\",\"sid\":\"388\"}},\"rhs\":{\"type\":\"tile\",\"args\":[{\"type\":\"evaluable\",\"expr\":\"28\",\"value\":28},{\"type\":\"evaluable\",\"expr\":\"1\",\"value\":1}]},\"equality\":true}"
      KernelAllAttrs=|
      | s[12;12;9;9;19;14;21;23;21;23;24;21;15;17;12;24;26;26;26;27;28;9;21;23;23;23;24;25;14;19;19;29]@FunctionNameDeclFileNamePortNamesPortTypesPortSerializedTypesPortDirectionsPortWindowSizeEnablesPortWindowMarginEnablesPortBufferSizeEnablesPortBufferMarginEnablesPortSynchronicityEnablesPortSignalSizeEnablesPortBufferSizesPortBufferMarginsFunctionDeclFunctionTemplateSpecKindFunctionTemplateParamNamesFunctionTemplateParamKindsFunctionTemplateParamTypesFunctionTemplateParamValuesFunctionTemplateParamEnablesClassDeclClassTemplateSpecKindClassTemplateParamNamesClassTemplateParamKindsClassTemplateParamTypesClassTemplateParamValuesClassTemplateParamEnablesClassCtorDeclsClassCtorParamNamesClassCtorParamTypesClassCtorParamSerializedTypes[1 1]@C[32 1]@t6@filtert39@../../src/aie_kernels/FirSingleStream.hC[2 1]@t3@sint4@coutC[2 1]@t21@input_stream_cint16 *t32@output_cascade< cacc48, void > *C[2 1]@t33@{P{Tinput_stream{1{t{Scint16}}}}}t42@{P{Toutput_cascade{2{t{Scacc48}}{t{Bv}}}}}C[2 1]@t5@inputt6@outputC[2 1]@l0@l0@C[2 1]@l0@l0@C[2 1]@l0@l0@C[2 1]@l0@l0@C[2 1]@l0@l0@C[2 1]@l0@l1@C[2 1]@nnC[2 1]@nnt169@namespace SingleStream {
      | template < int NSamples, int ShiftAcc > 
      | void FIR_MultiKernel_cout::
      | filter(input_stream_cint16 * sin, output_cascade< cacc48, void > * cout);
      | }t4@nonee[0 1]@e[0 1]@e[0 1]@e[0 1]@e[0 1]@t94@namespace SingleStream {
      | template < int NSamples, int ShiftAcc > class FIR_MultiKernel_cout;
      | }t8@implicitC[2 1]@t8@NSamplest8@ShiftAccC[2 1]@t7@nontypet7@nontypeC[2 1]@t3@intt3@intC[2 1]@nnC[2 1]@l1@l1@C[1 1]@t70@FIR_MultiKernel_cout(cint16 const ( & taps ) [ 8 ], int32 const Delay)C[1 1]@C[2 1]@t4@tapst5@DelayC[1 1]@C[2 1]@t23@cint16 const ( &) [ 8 ]t11@int32 constC[1 1]@C[2 1]@t20@{R{Q1{C{Scint16}8}}}t10@{Q1{Bi32}}
      FunctionDecl=|
      | namespace SingleStream {
      | template < int NSamples, int ShiftAcc > 
      | void FIR_MultiKernel_cout::
      | filter(input_stream_cint16 * sin, output_cascade< cacc48, void > * cout);
      | }
      ClassDeclTypeOptions=|
      | C[1 1]@t94@namespace SingleStream {
      | template < int NSamples, int ShiftAcc > class FIR_MultiKernel_cout;
      | }
      ClassDecl=|
      | namespace SingleStream {
      | template < int NSamples, int ShiftAcc > class FIR_MultiKernel_cout;
      | }
  Kernel_32 : aieBasic/AIE Class Kernel  KernelAllAttrs=|  PortNames={'sin'; 'cin'; 'sout'}  PortSerializedTypes={'{P{Tinput_stream{1{t{Scint16}}}}}'; '{P{Tinput_cascade{2{t{Scacc48}}{t{Bv}}}}}'; '{P{Toutput_stream{1{t{Scint16}}}}}'}  PortWindowSizes={0.000000000000000000e+00; 0.000000000000000000e+00; 0.000000000000000000e+00}  PortWindowMargins={0.000000000000000000e+00; 0.000000000000000000e+00; 0.000000000000000000e+00}  PortSynchronicities={'auto', 'auto', 'auto'}  PortSignalSizes={0.000000000000000000e+00; 0.000000000000000000e+00; 5.120000000000000000e+02}  ClassTemplateSpecKind=implicit  ClassTemplateParamNames={'NSamples'; 'ShiftAcc'}  ClassTemplateParamKinds={'nontype'; 'nontype'}  ClassTemplateParamTypes={'int'; 'int'}  ClassTemplateParamValues={'512', '15'}  ClassCtorParamNames={'taps'; 'Delay'}  ClassCtorParamSerializedTypes={'{R{Q1{C{Scint16}8}}}'; '{Q1{Bi32}}'}  ClassCtorParamValues={'[-83+21i -160-111i 237+54i 248+2878i 4086-5221i 1183-239i 146+91i -21-26i]', '0'}  ClassIndex=1  ClassCtorIndex=1  ClassTabVisible=on  ClassTemplateParamsVisible=on  ClassCtorDeclVisible=on  ClassCtorParamsVisible=on  FunctionTabVisible=on  FunctionDecl=|  PortAttrs={ 'input', 'sin', 'input_stream_cint16 *', '', '0', '', ''; 'input', 'cin', 'input_cascade< cacc48, void > *', '', '0', '', ''; 'output', 'sout', 'output_stream_cint16 *', '', '', '', 'N' }  PortAttrsEnables={'off', 'off', 'off', 'off', 'off', 'off', 'off';'off', 'off', 'off', 'off', 'off', 'off', 'off';'off', 'off', 'off', 'off', 'off', 'off', 'on'}  SampleTime=-1  ClassDeclTypeOptions=|  ClassDecl=|  ClassTemplateParams={ 'NSamples', 'int', 'BURST_LENGTH'; 'ShiftAcc', 'int', 'SHIFT_ACC' }  ClassTemplateParamsEnables={'off', 'off', 'on';'off', 'off', 'on'}  ClassCtorDeclTypeOptions=C[1 1]@t69@FIR_MultiKernel_cin(cint16 const ( & taps ) [ 8 ], int32 const Delay)  ClassCtorDecl=FIR_MultiKernel_cin(cint16 const ( & taps ) [ 8 ], int32 const Delay)  ClassCtorParams={ 'taps', 'cint16 const ( &) [ 8 ]', 'phi_1'; 'Delay', 'int32 const', '0' }  KernelHeaderFile=FirSingleStream.h  KernelClassName=SingleStream::FIR_MultiKernel_cin  KernelFunction=filter  KernelSourceFile=FirSingleStream.cpp  KernelSearchPaths={'$SRC', '$SRC/aie_kernels'}  PreProcOptions={}  blockJsonConstraints=[]
      KernelAllAttrs=|
      | s[12;12;9;9;19;14;21;23;21;23;24;21;15;17;12;24;26;26;26;27;28;9;21;23;23;23;24;25;14;19;19;29]@FunctionNameDeclFileNamePortNamesPortTypesPortSerializedTypesPortDirectionsPortWindowSizeEnablesPortWindowMarginEnablesPortBufferSizeEnablesPortBufferMarginEnablesPortSynchronicityEnablesPortSignalSizeEnablesPortBufferSizesPortBufferMarginsFunctionDeclFunctionTemplateSpecKindFunctionTemplateParamNamesFunctionTemplateParamKindsFunctionTemplateParamTypesFunctionTemplateParamValuesFunctionTemplateParamEnablesClassDeclClassTemplateSpecKindClassTemplateParamNamesClassTemplateParamKindsClassTemplateParamTypesClassTemplateParamValuesClassTemplateParamEnablesClassCtorDeclsClassCtorParamNamesClassCtorParamTypesClassCtorParamSerializedTypes[1 1]@C[32 1]@t6@filtert39@../../src/aie_kernels/FirSingleStream.hC[3 1]@t3@sint3@cint4@soutC[3 1]@t21@input_stream_cint16 *t31@input_cascade< cacc48, void > *t22@output_stream_cint16 *C[3 1]@t33@{P{Tinput_stream{1{t{Scint16}}}}}t41@{P{Tinput_cascade{2{t{Scacc48}}{t{Bv}}}}}t34@{P{Toutput_stream{1{t{Scint16}}}}}C[3 1]@t5@inputt5@inputt6@outputC[3 1]@l0@l0@l0@C[3 1]@l0@l0@l0@C[3 1]@l0@l0@l0@C[3 1]@l0@l0@l0@C[3 1]@l0@l0@l0@C[3 1]@l0@l0@l1@C[3 1]@nnnC[3 1]@nnnt195@namespace SingleStream {
      | template < int NSamples, int ShiftAcc > 
      | void FIR_MultiKernel_cin::
      | filter(input_stream_cint16 * sin, input_cascade< cacc48, void > * cin, output_stream_cint16 * sout);
      | }t4@nonee[0 1]@e[0 1]@e[0 1]@e[0 1]@e[0 1]@t93@namespace SingleStream {
      | template < int NSamples, int ShiftAcc > class FIR_MultiKernel_cin;
      | }t8@implicitC[2 1]@t8@NSamplest8@ShiftAccC[2 1]@t7@nontypet7@nontypeC[2 1]@t3@intt3@intC[2 1]@nnC[2 1]@l1@l1@C[1 1]@t69@FIR_MultiKernel_cin(cint16 const ( & taps ) [ 8 ], int32 const Delay)C[1 1]@C[2 1]@t4@tapst5@DelayC[1 1]@C[2 1]@t23@cint16 const ( &) [ 8 ]t11@int32 constC[1 1]@C[2 1]@t20@{R{Q1{C{Scint16}8}}}t10@{Q1{Bi32}}
      FunctionDecl=|
      | namespace SingleStream {
      | template < int NSamples, int ShiftAcc > 
      | void FIR_MultiKernel_cin::
      | filter(input_stream_cint16 * sin, input_cascade< cacc48, void > * cin, output_stream_cint16 * sout);
      | }
      ClassDeclTypeOptions=|
      | C[1 1]@t93@namespace SingleStream {
      | template < int NSamples, int ShiftAcc > class FIR_MultiKernel_cin;
      | }
      ClassDecl=|
      | namespace SingleStream {
      | template < int NSamples, int ShiftAcc > class FIR_MultiKernel_cin;
      | }
  Kernel_33 : aieBasic/AIE Class Kernel  KernelAllAttrs=|  PortNames={'sin'; 'cout'}  PortSerializedTypes={'{P{Tinput_stream{1{t{Scint16}}}}}'; '{P{Toutput_cascade{2{t{Scacc48}}{t{Bv}}}}}'}  PortWindowSizes={0.000000000000000000e+00; 0.000000000000000000e+00}  PortWindowMargins={0.000000000000000000e+00; 0.000000000000000000e+00}  PortSynchronicities={'auto', 'auto'}  PortSignalSizes={0.000000000000000000e+00; 5.120000000000000000e+02}  ClassTemplateSpecKind=implicit  ClassTemplateParamNames={'NSamples'; 'ShiftAcc'}  ClassTemplateParamKinds={'nontype'; 'nontype'}  ClassTemplateParamTypes={'int'; 'int'}  ClassTemplateParamValues={'512', '15'}  ClassCtorParamNames={'taps'; 'Delay'}  ClassCtorParamSerializedTypes={'{R{Q1{C{Scint16}8}}}'; '{Q1{Bi32}}'}  ClassCtorParamValues={'[-54-21i -121-233i 102-525i 237-96i 8773-2748i 1454+497i 342+439i 14+121i]', '0'}  ClassIndex=1  ClassCtorIndex=1  ClassTabVisible=on  ClassTemplateParamsVisible=on  ClassCtorDeclVisible=on  ClassCtorParamsVisible=on  FunctionTabVisible=on  FunctionDecl=|  PortAttrs={ 'input', 'sin', 'input_stream_cint16 *', '', '0', '', ''; 'output', 'cout', 'output_cascade< cacc48, void > *', '', '', '', 'N' }  PortAttrsEnables={'off', 'off', 'off', 'off', 'off', 'off', 'off';'off', 'off', 'off', 'off', 'off', 'off', 'on'}  SampleTime=-1  ClassDeclTypeOptions=|  ClassDecl=|  ClassTemplateParams={ 'NSamples', 'int', 'BURST_LENGTH'; 'ShiftAcc', 'int', 'SHIFT_ACC' }  ClassTemplateParamsEnables={'off', 'off', 'on';'off', 'off', 'on'}  ClassCtorDeclTypeOptions=C[1 1]@t70@FIR_MultiKernel_cout(cint16 const ( & taps ) [ 8 ], int32 const Delay)  ClassCtorDecl=FIR_MultiKernel_cout(cint16 const ( & taps ) [ 8 ], int32 const Delay)  ClassCtorParams={ 'taps', 'cint16 const ( &) [ 8 ]', 'phi_0'; 'Delay', 'int32 const', '0' }  KernelHeaderFile=FirSingleStream.h  KernelClassName=SingleStream::FIR_MultiKernel_cout  KernelFunction=filter  KernelSourceFile=FirSingleStream.cpp  KernelSearchPaths={'$SRC', '$SRC/aie_kernels'}  PreProcOptions={}  blockJsonConstraints="{\"type\":\"constraint\",\"constraintType\":\"location_kernel\",\"sid\":\"387\",\"lhs\":{\"type\":\"location\",\"templParam\":\"kernel\",\"args\":{\"type\":\"kernel\",\"name\":\"SingleStreamSSR/SSR4/Kernel_33\",\"sid\":\"387\"}},\"rhs\":{\"type\":\"tile\",\"args\":[{\"type\":\"evaluable\",\"expr\":\"28\",\"value\":28},{\"type\":\"evaluable\",\"expr\":\"3\",\"value\":3}]},\"equality\":true}"
      KernelAllAttrs=|
      | s[12;12;9;9;19;14;21;23;21;23;24;21;15;17;12;24;26;26;26;27;28;9;21;23;23;23;24;25;14;19;19;29]@FunctionNameDeclFileNamePortNamesPortTypesPortSerializedTypesPortDirectionsPortWindowSizeEnablesPortWindowMarginEnablesPortBufferSizeEnablesPortBufferMarginEnablesPortSynchronicityEnablesPortSignalSizeEnablesPortBufferSizesPortBufferMarginsFunctionDeclFunctionTemplateSpecKindFunctionTemplateParamNamesFunctionTemplateParamKindsFunctionTemplateParamTypesFunctionTemplateParamValuesFunctionTemplateParamEnablesClassDeclClassTemplateSpecKindClassTemplateParamNamesClassTemplateParamKindsClassTemplateParamTypesClassTemplateParamValuesClassTemplateParamEnablesClassCtorDeclsClassCtorParamNamesClassCtorParamTypesClassCtorParamSerializedTypes[1 1]@C[32 1]@t6@filtert39@../../src/aie_kernels/FirSingleStream.hC[2 1]@t3@sint4@coutC[2 1]@t21@input_stream_cint16 *t32@output_cascade< cacc48, void > *C[2 1]@t33@{P{Tinput_stream{1{t{Scint16}}}}}t42@{P{Toutput_cascade{2{t{Scacc48}}{t{Bv}}}}}C[2 1]@t5@inputt6@outputC[2 1]@l0@l0@C[2 1]@l0@l0@C[2 1]@l0@l0@C[2 1]@l0@l0@C[2 1]@l0@l0@C[2 1]@l0@l1@C[2 1]@nnC[2 1]@nnt169@namespace SingleStream {
      | template < int NSamples, int ShiftAcc > 
      | void FIR_MultiKernel_cout::
      | filter(input_stream_cint16 * sin, output_cascade< cacc48, void > * cout);
      | }t4@nonee[0 1]@e[0 1]@e[0 1]@e[0 1]@e[0 1]@t94@namespace SingleStream {
      | template < int NSamples, int ShiftAcc > class FIR_MultiKernel_cout;
      | }t8@implicitC[2 1]@t8@NSamplest8@ShiftAccC[2 1]@t7@nontypet7@nontypeC[2 1]@t3@intt3@intC[2 1]@nnC[2 1]@l1@l1@C[1 1]@t70@FIR_MultiKernel_cout(cint16 const ( & taps ) [ 8 ], int32 const Delay)C[1 1]@C[2 1]@t4@tapst5@DelayC[1 1]@C[2 1]@t23@cint16 const ( &) [ 8 ]t11@int32 constC[1 1]@C[2 1]@t20@{R{Q1{C{Scint16}8}}}t10@{Q1{Bi32}}
      FunctionDecl=|
      | namespace SingleStream {
      | template < int NSamples, int ShiftAcc > 
      | void FIR_MultiKernel_cout::
      | filter(input_stream_cint16 * sin, output_cascade< cacc48, void > * cout);
      | }
      ClassDeclTypeOptions=|
      | C[1 1]@t94@namespace SingleStream {
      | template < int NSamples, int ShiftAcc > class FIR_MultiKernel_cout;
      | }
      ClassDecl=|
      | namespace SingleStream {
      | template < int NSamples, int ShiftAcc > class FIR_MultiKernel_cout;
      | }
  PLIO_I{0..3} (4 alike) : aieBasic/PLIO  PlioWidth=64  PlioFreqSpec=off  PlioFreq=250  ColLocation=0  channel=0  blockJsonConstraints=[]  deprecateConstraints=0
  PLIO_O{0..3} (4 alike) : aieBasic/PLIO  PlioWidth=64  PlioFreqSpec=off  PlioFreq=250  ColLocation=0  channel=0  blockJsonConstraints=[]  deprecateConstraints=0
  PhaseOut0 : Outport
  PhaseOut1 : Outport  Port=2
  PhaseOut2 : Outport  Port=3
  PhaseOut3 : Outport  Port=4
  wires:
  Kernel_22/1 -> Kernel_32/2
  Kernel_33/1 -> Kernel_23/2
  Kernel_21/1 -> Kernel_11/2
  Kernel_13/1 -> Kernel_03/2
  Kernel_02/1 -> Kernel_12/2
  Kernel_31/1 -> Kernel_21/2
  Kernel_23/1 -> Kernel_13/2
  Kernel_00/1 -> Kernel_10/2
  Kernel_10/1 -> Kernel_20/2
  Kernel_12/1 -> Kernel_22/2
  Kernel_11/1 -> Kernel_01/2
  Kernel_20/1 -> Kernel_30/2
  Kernel_03/1 -> PLIO_O3/1
  PLIO_O3/1 -> PhaseOut3/1
  FIFO_00/1 -> Kernel_00/1
  FIFO_02/1 -> Kernel_02/1
  FIFO_03/1 -> Kernel_03/1
  FIFO_01/1 -> Kernel_01/1
  FIFO_10/1 -> Kernel_10/1
  FIFO_12/1 -> Kernel_12/1
  FIFO_11/1 -> Kernel_11/1
  FIFO_13/1 -> Kernel_13/1
  FIFO_20/1 -> Kernel_20/1
  FIFO_22/1 -> Kernel_22/1
  FIFO_23/1 -> Kernel_23/1
  FIFO_21/1 -> Kernel_21/1
  FIFO_30/1 -> Kernel_30/1
  FIFO_32/1 -> Kernel_32/1
  FIFO_33/1 -> Kernel_33/1
  FIFO_31/1 -> Kernel_31/1
  Kernel_01/1 -> PLIO_O1/1
  PLIO_O1/1 -> PhaseOut1/1
  PhaseIn0_0/1 -> PLIO_I0/1
  PLIO_I0/1 -> FIFO_01/1, FIFO_03/1, FIFO_02/1, FIFO_00/1
  PhaseIn1_0/1 -> PLIO_I1/1
  PLIO_I1/1 -> FIFO_11/1, FIFO_13/1, FIFO_10/1, FIFO_12/1
  PhaseIn2_0/1 -> PLIO_I2/1
  PLIO_I2/1 -> FIFO_21/1, FIFO_23/1, FIFO_20/1, FIFO_22/1
  PhaseIn3_0/1 -> PLIO_I3/1
  PLIO_I3/1 -> FIFO_30/1, FIFO_32/1, FIFO_31/1, FIFO_33/1
  Kernel_32/1 -> PLIO_O2/1
  PLIO_O2/1 -> PhaseOut2/1
  Kernel_30/1 -> PLIO_O0/1
  PLIO_O0/1 -> PhaseOut0/1
